simulink library "xbsIndex_r4"  (Simulink 7.1)
(part 2 of 9)

      | patch([3 131 131 3 3 ],[0 0 165 165 0 ],[7.700000e-001 8.200000e-001 9.100000e-001 ]);
      | plot([3 131 131 3 3 ],[0 0 165 165 0 ]);
      | 
      | 
      | patch([24.725 52.18 71.18 90.18 109.18 71.18 43.725 24.725 ],[103.09 103.09 122.09 103.09 122.09 122.09 122.09 103.09 ],[1 1 1 ]);
      | patch([43.725 71.18 52.18 24.725 43.725 ],[84.09 84.09 103.09 103.09 84.09 ],[0.931 0.946 0.973 ]);
      | patch([24.725 52.18 71.18 43.725 24.725 ],[65.09 65.09 84.09 84.09 65.09 ],[1 1 1 ]);
      | patch([43.725 109.18 90.18 71.18 52.18 24.725 43.725 ],[46.09 46.09 65.09 46.09 65.09 65.09 46.09 ],[0.931 0.946 0.973 ]);
      | fprintf('','COMMENT: end icon graphics');
      | fprintf('','COMMENT: begin icon text');
      | color('black');port_label('input',1,'  a_tvalid  ');
      | color('black');port_label('input',2,'  a_tdata_imag  ');
      | color('black');port_label('input',3,'  a_tdata_real  ');
      | color('black');port_label('input',4,'  b_tvalid  ');
      | color('black');port_label('input',5,'  b_tdata_imag  ');
      | color('black');port_label('input',6,'  b_tdata_real  ');
      | color('black');port_label('output',1,'  dout_tvalid  ');
      | color('black');port_label('output',2,'  dout_tdata_imag  ');
      | color('black');port_label('output',3,'  dout_tdata_real  ');
      | fprintf('','COMMENT: end icon text');
  "Complex Multiplier 5.0 " : S-Function  LoadFcn=xlBlockLoadCallback(gcbh);  FunctionName=sysgen  Parameters=ptable_  EnableBusSupport=off  mask(Xilinx Complex Multiplier 5.0  Block){hasatlast_sgadvanced=, hasatlast=off, hasatuser_sgadvanced=, hasatuser=off, atuserwidth=1, hasbtlast_sgadvanced=, hasbtlast=off, hasbtuser_sgadvanced=, hasbtuser=off, btuserwidth=1, multtype_sgadvanced=, multtype=Use_Mults, optimizegoal_sgadvanced=, optimizegoal=Resources, flowcontrol_sgadvanced=, flowcontrol=NonBlocking, outputwidth=33, roundmode_sgadvanced=, roundmode=Truncate, hasctrltlast_sgadvanced=, hasctrltlast=off, hasctrltuser_sgadvanced=, hasctrltuser=off, ctrltuserwidth=1, outtlastbehv=Null, latencyconfig=Automatic, minimumlatency=15, aclken_sgadvanced=, aclken=off, aresetn_sgadvanced=, aresetn=off, trim_axipin_name=on, aportwidth=63, bportwidth=63, ip_name=Complex Multiplier, ip_version=5.0, dsptool_ready=true, ipcore_usecache=true, ipcore_useipmodelcache=true, ipcore_verbose=false, ipcore_latency_parameter='minimumlatency', wrapper_available=true, port_translation_map={ 'aclken' => 'en', 'aresetn' => 'rst'}, structural_sim=false, has_advanced_control=0, sggui_pos=-1,-1,-1,-1, block_type=cmpy_v5_0, block_version=, sg_icon_stat=135,165,6,3,white,blue,0,7e63527f,right,,[2 2 2 3 3 3 ],[4 4 4 ], sg_mask_display=|, sg_list_contents=, sg_blockgui_xml=}
      mask sg_mask_display=|
      | fprintf('','COMMENT: begin icon graphics');
      | patch([0 0 3 3 ],[154 86 86 154 ],[6.025000e-001 6.400000e-001 7.075000e-001 ]);
      | patch([0 0 3 3 ],[79 11 11 79 ],[4.350000e-001 4.600000e-001 5.050000e-001 ]);
      | patch([132 132 135 135 ],[154 6 6 154 ],[2.675000e-001 2.800000e-001 3.025000e-001 ]);
      | patch([3 131 131 3 3 ],[0 0 165 165 0 ],[7.700000e-001 8.200000e-001 9.100000e-001 ]);
      | plot([3 131 131 3 3 ],[0 0 165 165 0 ]);
      |
      |
      | patch([24.725 52.18 71.18 90.18 109.18 71.18 43.725 24.725 ],[103.09 103.09 122.09 103.09 122.09 122.09 122.09 103.09 ],[1 1 1 ]);
      | patch([43.725 71.18 52.18 24.725 43.725 ],[84.09 84.09 103.09 103.09 84.09 ],[0.931 0.946 0.973 ]);
      | patch([24.725 52.18 71.18 43.725 24.725 ],[65.09 65.09 84.09 84.09 65.09 ],[1 1 1 ]);
      | patch([43.725 109.18 90.18 71.18 52.18 24.725 43.725 ],[46.09 46.09 65.09 46.09 65.09 65.09 46.09 ],[0.931 0.946 0.973 ]);
      | fprintf('','COMMENT: end icon graphics');
      | fprintf('','COMMENT: begin icon text');
      | color('black');port_label('input',1,'  a_tvalid  ');
      | color('black');port_label('input',2,'  a_tdata_imag  ');
      | color('black');port_label('input',3,'  a_tdata_real  ');
      | color('black');port_label('input',4,'  b_tvalid  ');
      | color('black');port_label('input',5,'  b_tdata_imag  ');
      | color('black');port_label('input',6,'  b_tdata_real  ');
      | color('black');port_label('output',1,'  dout_tvalid  ');
      | color('black');port_label('output',2,'  dout_tdata_imag  ');
      | color('black');port_label('output',3,'  dout_tdata_real  ');
      | fprintf('','COMMENT: end icon text');
      mask prompts: hasatlast_sgadvanced ""; hasatlast "Has TLAST"; hasatuser_sgadvanced ""; hasatuser "Has TUSER"; atuserwidth "TUSER Width"; hasbtlast_sgadvanced ""; hasbtlast "Has TLAST"; hasbtuser_sgadvanced ""; hasbtuser "Has TUSER"; btuserwidth "TUSER Width"; multtype_sgadvanced ""; multtype ""; optimizegoal_sgadvanced ""; optimizegoal ""; flowcontrol_sgadvanced ""; flowcontrol ""; outputwidth "Output Width"; roundmode_sgadvanced ""; roundmode ""; hasctrltlast_sgadvanced ""; hasctrltlast "Has TLAST"; hasctrltuser_sgadvanced ""; hasctrltuser "Has TUSER"; ctrltuserwidth "TUSER Width"; outtlastbehv "TLAST Behavior"; latencyconfig "Latency Configuration"; minimumlatency "Minimum Latency"; aclken_sgadvanced ""; aresetn_sgadvanced ""; trim_axipin_name "Display shortened port names"; aportwidth ""; bportwidth ""; ip_name ""; ip_version ""; dsptool_ready ""; ipcore_usecache ""; ipcore_useipmodelcache ""; ipcore_verbose ""; ipcore_latency_parameter ""; wrapper_available ""; port_translation_map ""; structural_sim ""; has_advanced_control ""; sggui_pos ""; block_type ""; block_version ""; sg_icon_stat ""; sg_mask_display ""; sg_list_contents ""; sg_blockgui_xml ""
      mask help: Xilinx Complex Multiplier 5.0
      mask init:
      | try
      |   tmp_gcb = gcb;
      |   tmp_gcbh = gcbh;
      |   if (strcmp('SysGenIndex',get_param(bdroot(tmp_gcbh),'tag')) && ~isempty(regexp(bdroot(tmp_gcb), '^xbs', 'once')))
      |     return;
      |   end;
      |   xlMungeMaskParams;
      |   block_config = 'sysgen:coregenimport_config';
      | 
      |   block_type='cmpy_v5_0';
      | 
      |   serialized_declarations = '{''aclken''=>''Bool'',''aportwidth''=>''String'',''aresetn''=>''Bool'',''atuserwidth''=>''Int'',''bportwidth''=>''String'',''btuserwidth''=>''Int'',''ctrltuserwidth''=>''Int'',''dsptool_ready''=>''Bool'',''flowcontrol''=>''String'',''hasatlast''=>''Bool'',''hasatuser''=>''Bool'',''hasbtlast''=>''Bool'',''hasbtuser''=>''Bool'',''hasctrltlast''=>''Bool'',''hasctrltuser''=>''Bool'',''ip_name''=>''String'',''ip_version''=>''String'',''ipcore_latency_parameter''=>''String'',''ipcore_usecache''=>''Bool'',''ipcore_useipmodelcache''=>''Bool'',''ipcore_verbose''=>''Bool'',''latencyconfig''=>''String'',''minimumlatency''=>''Int'',''multtype''=>''String'',''optimizegoal''=>''String'',''outputwidth''=>''Int'',''outtlastbehv''=>''String'',''port_translation_map''=>''String'',''roundmode''=>''String'',''structural_sim''=>''Bool'',''trim_axipin_name''=>''Int'',''wrapper_available''=>''Bool'',''block_type''=>''String''}';
      |   ptable_ = xlblockprep(get_param(tmp_gcb, 'MaskWSVariables'));
      |   try
      |     xlBlockMoveCallback(tmp_gcbh);
      |   catch 
      |      clear global xl_updateicon_recursion_guard;
      |   end;
      | catch
      |   global dbgsysgen;
      |   if(~isempty(dbgsysgen) && dbgsysgen)
      |     e = regexprep(lasterr, '\n', '\nError: ');
      |     disp(['Error: While running MaskInit code on block ' tmp_gcb ': ' e]);
      |     error(e);
      |   end
      | end
      settings: CopyFcn=xlBlockMoveCallback(gcbh);  DeleteFcn=xlDestroyGui(gcbh);  ModelCloseFcn=xlDestroyGui(gcbh);  PreSaveFcn=xlBlockPreSaveCallback(gcbh);  PostSaveFcn=xlBlockPostSaveCallback(gcbh);  DestroyFcn=xlDestroyGui(gcbh);  OpenFcn=xlOpenGui(gcbh, 'cmpy_v5_0_gui.xml', @xlipmagiccallback_pass_evaluate_params, @xlipmagicaction)  CloseFcn=xlDestroyGui(gcbh);  MoveFcn=xlBlockMoveCallback(gcbh);
      mask Help: eval('');xlDoc('-book','sysgen','-topic','Complex_Multiplier_5_0');
      mask StyleString: edit,checkbox,edit,checkbox,edit,edit,checkbox,edit,checkbox,edit,edit,popup(Use_Mults|Use_LUTs),edit,popup(Resources|Performance),edit,popup(Blocking|NonBlocking),edit,edit,popup(Truncate|Random_Rounding),edit,checkbox,edit,checkbox,edit,popup(Null|Pass_A_TLAST|Pass_B_TLAST|Pass_CTRL_TLAST|OR_all_TLASTs|AND_all_TLASTs),popup(Automatic|Manual),edit,edit,checkbox,edit,checkbox,checkbox,edit,edit,edit,edit,edit,edit,edit,edit,edit,edit,edit,edit,edit,edit,edit,edit,edit,edit,edit,edit
      mask Display:
      | fprintf('','COMMENT: begin icon graphics');
      | patch([0 0 3 3 ],[154 86 86 154 ],[6.025000e-001 6.400000e-001 7.075000e-001 ]);
      | patch([0 0 3 3 ],[79 11 11 79 ],[4.350000e-001 4.600000e-001 5.050000e-001 ]);
      | patch([132 132 135 135 ],[154 6 6 154 ],[2.675000e-001 2.800000e-001 3.025000e-001 ]);
      | patch([3 131 131 3 3 ],[0 0 165 165 0 ],[7.700000e-001 8.200000e-001 9.100000e-001 ]);
      | plot([3 131 131 3 3 ],[0 0 165 165 0 ]);
      | 
      | 
      | patch([24.725 52.18 71.18 90.18 109.18 71.18 43.725 24.725 ],[103.09 103.09 122.09 103.09 122.09 122.09 122.09 103.09 ],[1 1 1 ]);
      | patch([43.725 71.18 52.18 24.725 43.725 ],[84.09 84.09 103.09 103.09 84.09 ],[0.931 0.946 0.973 ]);
      | patch([24.725 52.18 71.18 43.725 24.725 ],[65.09 65.09 84.09 84.09 65.09 ],[1 1 1 ]);
      | patch([43.725 109.18 90.18 71.18 52.18 24.725 43.725 ],[46.09 46.09 65.09 46.09 65.09 65.09 46.09 ],[0.931 0.946 0.973 ]);
      | fprintf('','COMMENT: end icon graphics');
      | fprintf('','COMMENT: begin icon text');
      | color('black');port_label('input',1,'  a_tvalid  ');
      | color('black');port_label('input',2,'  a_tdata_imag  ');
      | color('black');port_label('input',3,'  a_tdata_real  ');
      | color('black');port_label('input',4,'  b_tvalid  ');
      | color('black');port_label('input',5,'  b_tdata_imag  ');
      | color('black');port_label('input',6,'  b_tdata_real  ');
      | color('black');port_label('output',1,'  dout_tvalid  ');
      | color('black');port_label('output',2,'  dout_tdata_imag  ');
      | color('black');port_label('output',3,'  dout_tdata_real  ');
      | fprintf('','COMMENT: end icon text');
  Concat : S-Function  LoadFcn=xlBlockLoadCallback(gcbh);  FunctionName=sysgen  Parameters=ptable_  EnableBusSupport=off  mask(Xilinx Bus Concatenator Block){infoedit=Concatenates two or more inputs.  Output will be cast to an unsigned value with the binary point at zero., num_inputs=2, dbl_ovrd_sgadvanced=, dbl_ovrd=off, has_advanced_control=0, sggui_pos=-1,-1,-1,-1, block_type=concat, block_version=, sg_icon_stat=60,60,2,1,white,blue,0,16398980,right,,[ ],[ ], sg_mask_display=|, sg_list_contents=, sg_blockgui_xml=}
      mask sg_mask_display=|
      | fprintf('','COMMENT: begin icon graphics');
      | patch([0 60 60 0 0 ],[0 0 60 60 0 ],[0.77 0.82 0.91 ]);
      | plot([0 60 60 0 0 ],[0 0 60 60 0 ]);
      | patch([12.2 23.76 31.76 39.76 47.76 31.76 20.2 12.2 ],[38.88 38.88 46.88 38.88 46.88 46.88 46.88 38.88 ],[1 1 1 ]);
      | patch([20.2 31.76 23.76 12.2 20.2 ],[30.88 30.88 38.88 38.88 30.88 ],[0.931 0.946 0.973 ]);
      | patch([12.2 23.76 31.76 20.2 12.2 ],[22.88 22.88 30.88 30.88 22.88 ],[1 1 1 ]);
      | patch([20.2 47.76 39.76 31.76 23.76 12.2 20.2 ],[14.88 14.88 22.88 14.88 22.88 22.88 14.88 ],[0.931 0.946 0.973 ]);
      | fprintf('','COMMENT: end icon graphics');
      | fprintf('','COMMENT: begin icon text');
      | color('black');port_label('input',1,'hi');
      | color('black');port_label('input',2,'lo');
      |
      | color('black');disp('\fontsize{20}\}','texmode','on');
      | fprintf('','COMMENT: end icon text');
      mask prompts: infoedit ""; num_inputs "Number of inputs"; dbl_ovrd_sgadvanced ""; dbl_ovrd "Override with doubles"; has_advanced_control ""; sggui_pos ""; block_type ""; block_version ""; sg_icon_stat ""; sg_mask_display ""; sg_list_contents ""; sg_blockgui_xml ""
      mask help: Concatenates two or more inputs. Output will be cast to an unsigned value with the binary point at zero.
      mask init:
      | try
      |   tmp_gcb = gcb;
      |   tmp_gcbh = gcbh;
      |   if (strcmp('SysGenIndex',get_param(bdroot(tmp_gcbh),'tag')) && ~isempty(regexp(bdroot(tmp_gcb), '^xbs', 'once')))
      |     return;
      |   end;
      |   xlMungeMaskParams;
      |   block_config = 'sysgen_blockset:Concat_config';
      | 
      |   block_type='concat';
      | 
      |   serialized_declarations = '{''num_inputs''=>''Int'',''sim_engine''=>''Int'',''sysgen_root''=>''String'',''block_type''=>''String''}';
      |   xlconcat_init();
      |   ptable_ = xlblockprep(get_param(tmp_gcb, 'MaskWSVariables'));
      |   try
      |     xlBlockMoveCallback(tmp_gcbh);
      |   catch 
      |      clear global xl_updateicon_recursion_guard;
      |   end;
      | catch
      |   global dbgsysgen;
      |   if(~isempty(dbgsysgen) && dbgsysgen)
      |     e = regexprep(lasterr, '\n', '\nError: ');
      |     disp(['Error: While running MaskInit code on block ' tmp_gcb ': ' e]);
      |     error(e);
      |   end
      | end
      settings: CopyFcn=xlBlockMoveCallback(gcbh);  DeleteFcn=xlDestroyGui(gcbh);  ModelCloseFcn=xlDestroyGui(gcbh);  PreSaveFcn=xlBlockPreSaveCallback(gcbh);  PostSaveFcn=xlBlockPostSaveCallback(gcbh);  DestroyFcn=xlDestroyGui(gcbh);  OpenFcn=xlOpenGui(gcbh, 'concat_gui.xml', @xlmagicenablement, -1)  CloseFcn=xlDestroyGui(gcbh);  MoveFcn=xlBlockMoveCallback(gcbh);
      mask Help: eval('');xlDoc('-book','sysgen','-topic','Concat');
      mask Display:
      | fprintf('','COMMENT: begin icon graphics');
      | patch([0 60 60 0 0 ],[0 0 60 60 0 ],[0.77 0.82 0.91 ]);
      | plot([0 60 60 0 0 ],[0 0 60 60 0 ]);
      | patch([12.2 23.76 31.76 39.76 47.76 31.76 20.2 12.2 ],[38.88 38.88 46.88 38.88 46.88 46.88 46.88 38.88 ],[1 1 1 ]);
      | patch([20.2 31.76 23.76 12.2 20.2 ],[30.88 30.88 38.88 38.88 30.88 ],[0.931 0.946 0.973 ]);
      | patch([12.2 23.76 31.76 20.2 12.2 ],[22.88 22.88 30.88 30.88 22.88 ],[1 1 1 ]);
      | patch([20.2 47.76 39.76 31.76 23.76 12.2 20.2 ],[14.88 14.88 22.88 14.88 22.88 22.88 14.88 ],[0.931 0.946 0.973 ]);
      | fprintf('','COMMENT: end icon graphics');
      | fprintf('','COMMENT: begin icon text');
      | color('black');port_label('input',1,'hi');
      | color('black');port_label('input',2,'lo');
      | 
      | color('black');disp('\fontsize{20}\}','texmode','on');
      | fprintf('','COMMENT: end icon text');
  Configurable Subsystem Manager : S-Function  Tag=xcfgMgr  FunctionName=xlpermissive  Parameters=''  EnableBusSupport=off  mask(Xilinx Configurable Subsystem Manager Block){infoedit=Configurable Subsystem Manager, ShowPortLabels=, has_advanced_control=0, sggui_pos=-1,-1,-1,-1, block_type=configurable_subsystem_manager, block_version=, sg_icon_stat=53,51,-1,-1,blue,white,0,07734,right,,[ ],[ ], sg_mask_display=|, sg_list_contents=, sg_blockgui_xml=}
      mask sg_mask_display=|
      | fprintf('','COMMENT: begin icon graphics');
      | patch([0 53 53 0 0 ],[0 0 51 51 0 ],[1 1 1 ]);
      | plot([0 53 53 0 0 ],[0 0 51 51 0 ]);
      | patch([10.425 20.54 27.54 34.54 41.54 27.54 17.425 10.425 ],[32.77 32.77 39.77 32.77 39.77 39.77 39.77 32.77 ],[0.839 0.874 0.937 ]);
      | patch([17.425 27.54 20.54 10.425 17.425 ],[25.77 25.77 32.77 32.77 25.77 ],[0.77 0.82 0.91 ]);
      | patch([10.425 20.54 27.54 17.425 10.425 ],[18.77 18.77 25.77 25.77 18.77 ],[0.839 0.874 0.937 ]);
      | patch([17.425 41.54 34.54 27.54 20.54 10.425 17.425 ],[11.77 11.77 18.77 11.77 18.77 18.77 11.77 ],[0.77 0.82 0.91 ]);
      | fprintf('','COMMENT: end icon graphics');
      | fprintf('','COMMENT: begin icon text');
      | fprintf('','COMMENT: end icon text');
      mask prompts: infoedit ""; ShowPortLabels ""; has_advanced_control ""; sggui_pos ""; block_type ""; block_version ""; sg_icon_stat ""; sg_mask_display ""; sg_list_contents ""; sg_blockgui_xml ""
      mask help: Configurable Subsystem Manager
      mask init:
      | try
      |   tmp_gcb = gcb;
      |   tmp_gcbh = gcbh;
      |   if (strcmp('SysGenIndex',get_param(bdroot(tmp_gcbh),'tag')) && ~isempty(regexp(bdroot(tmp_gcb), '^xbs', 'once')))
      |     return;
      |   end;
      |   xlMungeMaskParams;
      | 
      |   block_type='configurable_subsystem_manager';
      | 
      |   serialized_declarations = '{''block_type''=>''String''}';
      |   ptable_ = xlblockprep(get_param(tmp_gcb, 'MaskWSVariables'));
      |   try
      |     xlBlockMoveCallback(tmp_gcbh);
      |   catch 
      |      clear global xl_updateicon_recursion_guard;
      |   end;
      | catch
      |   global dbgsysgen;
      |   if(~isempty(dbgsysgen) && dbgsysgen)
      |     e = regexprep(lasterr, '\n', '\nError: ');
      |     disp(['Error: While running MaskInit code on block ' tmp_gcb ': ' e]);
      |     error(e);
      |   end
      | end
      settings: AttributesFormatString=Configurable Subsystem\nManager  CopyFcn=xlBlockMoveCallback(gcbh);  DeleteFcn=xlconfig_mgr_callback(gcb, 'DeleteFcn');  OpenFcn=xlconfig_mgr_callback(gcb, 'OpenFcn');  MoveFcn=xlBlockMoveCallback(gcbh);
      mask Help: eval('');xlDoc('-book','sysgen','-topic','Configurable_Subsystem_Manager');
      mask Display:
      | fprintf('','COMMENT: begin icon graphics');
      | patch([0 53 53 0 0 ],[0 0 51 51 0 ],[1 1 1 ]);
      | plot([0 53 53 0 0 ],[0 0 51 51 0 ]);
      | patch([10.425 20.54 27.54 34.54 41.54 27.54 17.425 10.425 ],[32.77 32.77 39.77 32.77 39.77 39.77 39.77 32.77 ],[0.839 0.874 0.937 ]);
      | patch([17.425 27.54 20.54 10.425 17.425 ],[25.77 25.77 32.77 32.77 25.77 ],[0.77 0.82 0.91 ]);
      | patch([10.425 20.54 27.54 17.425 10.425 ],[18.77 18.77 25.77 25.77 18.77 ],[0.839 0.874 0.937 ]);
      | patch([17.425 41.54 34.54 27.54 20.54 10.425 17.425 ],[11.77 11.77 18.77 11.77 18.77 18.77 11.77 ],[0.77 0.82 0.91 ]);
      | fprintf('','COMMENT: end icon graphics');
      | fprintf('','COMMENT: begin icon text');
      | fprintf('','COMMENT: end icon text');
  Constant : S-Function  LoadFcn=xlBlockLoadCallback(gcbh);  FunctionName=sysgen  Parameters=ptable_  EnableBusSupport=off  mask(Xilinx Constant Block Block){const=1, gui_display_data_type=Fixed-point, arith_type_sgadvanced=, arith_type=Signed (2's comp), n_bits=16, bin_pt=14, preci_type_sgadvanced=, preci_type=Single, exp_width=8, frac_width=24, explicit_period_sgadvanced=, explicit_period=off, period=1, dsp48_infoedit=The use of this block for DSP48 instructions is deprecated.  Please use the Opmode block., equ=P=C, opselect_sgadvanced=, opselect=C, inp2_sgadvanced=, inp2=PCIN>>17, opr_sgadvanced=, opr=+, inp1_sgadvanced=, inp1=P, carry_sgadvanced=, carry=CIN, dbl_ovrd_sgadvanced=, dbl_ovrd=off, has_advanced_control=0, sggui_pos=-1,-1,-1,-1, block_type=constant, block_version=, sg_icon_stat=55,26,0,1,white,blue,0,1c72b5be,right,,[ ],[ ], sg_mask_display=|, sg_list_contents=, sg_blockgui_xml=}
      mask sg_mask_display=|
      | fprintf('','COMMENT: begin icon graphics');
      | patch([0 55 55 0 0 ],[0 0 26 26 0 ],[0.77 0.82 0.91 ]);
      | plot([0 55 55 0 0 ],[0 0 26 26 0 ]);
      | patch([20.325 24.66 27.66 30.66 33.66 27.66 23.325 20.325 ],[16.33 16.33 19.33 16.33 19.33 19.33 19.33 16.33 ],[1 1 1 ]);
      | patch([23.325 27.66 24.66 20.325 23.325 ],[13.33 13.33 16.33 16.33 13.33 ],[0.931 0.946 0.973 ]);
      | patch([20.325 24.66 27.66 23.325 20.325 ],[10.33 10.33 13.33 13.33 10.33 ],[1 1 1 ]);
      | patch([23.325 33.66 30.66 27.66 24.66 20.325 23.325 ],[7.33 7.33 10.33 7.33 10.33 10.33 7.33 ],[0.931 0.946 0.973 ]);
      | fprintf('','COMMENT: end icon graphics');
      | fprintf('','COMMENT: begin icon text');
      | color('black');port_label('output',1,'1');
      | fprintf('','COMMENT: end icon text');
      mask prompts: const "Constant value"; gui_display_data_type ""; arith_type_sgadvanced ""; arith_type "Arithmetic type"; n_bits "Number of bits"; bin_pt "Binary point"; preci_type_sgadvanced ""; preci_type ""; exp_width "Exponent width"; frac_width "Fraction width"; explicit_period_sgadvanced ""; explicit_period "Sampled constant"; period "Sample period"; dsp48_infoedit ""; equ "DSP48 operation"; opselect_sgadvanced ""; opselect "Operation select"; inp2_sgadvanced ""; inp2 "Z mux"; opr_sgadvanced ""; opr "Operand"; inp1_sgadvanced ""; inp1 "YX muxes"; carry_sgadvanced ""; carry "Carry input"; dbl_ovrd_sgadvanced ""; dbl_ovrd "Override with doubles"; has_advanced_control ""; sggui_pos ""; block_type ""; block_version ""; sg_icon_stat ""; sg_mask_display ""; sg_list_contents ""; sg_blockgui_xml ""
      mask help: Xilinx Constant Block
      mask init:
      | try
      |   tmp_gcb = gcb;
      |   tmp_gcbh = gcbh;
      |   if (strcmp('SysGenIndex',get_param(bdroot(tmp_gcbh),'tag')) && ~isempty(regexp(bdroot(tmp_gcb), '^xbs', 'once')))
      |     return;
      |   end;
      |   xlMungeMaskParams;
      |   block_config = 'sysgen_blockset:Constant_config';
      | 
      |   block_type='constant';
      | 
      |   serialized_declarations = '{''arith_type''=>''Int'',''bin_pt''=>''Int'',''carry''=>''Int'',''const''=>''Double'',''dbl_ovrd''=>''Int'',''exp_width''=>''Int'',''explicit_period''=>''Int'',''frac_width''=>''Int'',''gui_display_data_type''=>''Int'',''inp1''=>''Int'',''inp2''=>''Int'',''n_bits''=>''Int'',''opr''=>''Int'',''opselect''=>''Int'',''period''=>''Double'',''preci_type''=>''Int'',''block_type''=>''String''}';
      |   xlconstant_init();
      |   ptable_ = xlblockprep(get_param(tmp_gcb, 'MaskWSVariables'));
      |   try
      |     xlBlockMoveCallback(tmp_gcbh);
      |   catch 
      |      clear global xl_updateicon_recursion_guard;
      |   end;
      | catch
      |   global dbgsysgen;
      |   if(~isempty(dbgsysgen) && dbgsysgen)
      |     e = regexprep(lasterr, '\n', '\nError: ');
      |     disp(['Error: While running MaskInit code on block ' tmp_gcb ': ' e]);
      |     error(e);
      |   end
      | end
      settings: CopyFcn=xlBlockMoveCallback(gcbh);  DeleteFcn=xlDestroyGui(gcbh);  ModelCloseFcn=xlDestroyGui(gcbh);  PreSaveFcn=xlBlockPreSaveCallback(gcbh);  PostSaveFcn=xlBlockPostSaveCallback(gcbh);  DestroyFcn=xlDestroyGui(gcbh);  OpenFcn=xlOpenGui(gcbh, 'constant_gui.xml', @constantenablement, @constantaction)  CloseFcn=xlDestroyGui(gcbh);  MoveFcn=xlBlockMoveCallback(gcbh);
      mask Help: eval('');xlDoc('-book','sysgen','-topic','Constant');
      mask StyleString: edit,popup(Boolean|Fixed-point|Floating-point),edit,popup(Boolean|Signed (2's comp)|Unsigned|DSP48 Instruction|Floating-point),edit,edit,edit,popup(Single|Double|Custom),edit,edit,edit,checkbox,edit,edit,edit,edit,popup(C + A*B|PCIN + A*B|P + A*B|A * B|C + A:B|C - A:B|C|Custom),edit,popup(0|PCIN|P|C|PCIN>>17|P>>17),edit,popup(+|-),edit,popup(0|P|A:B|A*B|C|P+C|A:B+C),edit,popup(0|1|CIN|~SIGN(P or PCIN)|~SIGN(A*B or A:B)|~SIGND(A*B or A:B)),edit,checkbox,edit,edit,edit,edit,edit,edit,edit,edit
      mask Display:
      | fprintf('','COMMENT: begin icon graphics');
      | patch([0 55 55 0 0 ],[0 0 26 26 0 ],[0.77 0.82 0.91 ]);
      | plot([0 55 55 0 0 ],[0 0 26 26 0 ]);
      | patch([20.325 24.66 27.66 30.66 33.66 27.66 23.325 20.325 ],[16.33 16.33 19.33 16.33 19.33 19.33 19.33 16.33 ],[1 1 1 ]);
      | patch([23.325 27.66 24.66 20.325 23.325 ],[13.33 13.33 16.33 16.33 13.33 ],[0.931 0.946 0.973 ]);
      | patch([20.325 24.66 27.66 23.325 20.325 ],[10.33 10.33 13.33 13.33 10.33 ],[1 1 1 ]);
      | patch([23.325 33.66 30.66 27.66 24.66 20.325 23.325 ],[7.33 7.33 10.33 7.33 10.33 10.33 7.33 ],[0.931 0.946 0.973 ]);
      | fprintf('','COMMENT: end icon graphics');
      | fprintf('','COMMENT: begin icon text');
      | color('black');port_label('output',1,'1');
      | fprintf('','COMMENT: end icon text');
  Convert : S-Function  LoadFcn=xlBlockLoadCallback(gcbh);  FunctionName=sysgen  Parameters=ptable_  EnableBusSupport=off  mask(Xilinx Type Converter Block){infoedit=Hardware notes: rounding and saturating require hardware resources; truncating and wrapping do not., gui_display_data_type_sgadvanced=, gui_display_data_type=Fixed-point, arith_type_sgadvanced=, arith_type=Signed  (2's comp), n_bits=16, bin_pt=14, float_type_sgadvanced=, float_type=Single, exp_bits=8, fraction_bits=24, quantization_sgadvanced=, quantization=Truncate, overflow_sgadvanced=, overflow=Wrap, en_sgadvanced=, en=off, latency=0, dbl_ovrd_sgadvanced=, dbl_ovrd=off, pipeline_sgadvanced=, pipeline=off, xl_use_area_sgadvanced=, xl_use_area=off, xl_area=[0,0,0,0,0,0,0], has_advanced_control=0, sggui_pos=-1,-1,-1,-1, block_type=convert, block_version=, sg_icon_stat=45,30,1,1,white,blue,0,edca21da,right,,[ ],[ ], sg_mask_display=|, sg_list_contents=, sg_blockgui_xml=}
      mask sg_mask_display=|
      | fprintf('','COMMENT: begin icon graphics');
      | patch([0 45 45 0 0 ],[0 0 30 30 0 ],[0.77 0.82 0.91 ]);
      | plot([0 45 45 0 0 ],[0 0 30 30 0 ]);
      | patch([13.1 18.88 22.88 26.88 30.88 22.88 17.1 13.1 ],[19.44 19.44 23.44 19.44 23.44 23.44 23.44 19.44 ],[1 1 1 ]);
      | patch([17.1 22.88 18.88 13.1 17.1 ],[15.44 15.44 19.44 19.44 15.44 ],[0.931 0.946 0.973 ]);
      | patch([13.1 18.88 22.88 17.1 13.1 ],[11.44 11.44 15.44 15.44 11.44 ],[1 1 1 ]);
      | patch([17.1 30.88 26.88 22.88 18.88 13.1 17.1 ],[7.44 7.44 11.44 7.44 11.44 11.44 7.44 ],[0.931 0.946 0.973 ]);
      | fprintf('','COMMENT: end icon graphics');
      | fprintf('','COMMENT: begin icon text');
      |
      | color('black');port_label('output',1,'cast');
      | fprintf('','COMMENT: end icon text');
      mask prompts: infoedit ""; gui_display_data_type_sgadvanced ""; gui_display_data_type ""; arith_type_sgadvanced ""; arith_type "Arithmetic type"; n_bits "Number of bits"; bin_pt "Binary point"; float_type_sgadvanced ""; float_type ""; exp_bits "Exponent width"; fraction_bits "Fraction width"; quantization_sgadvanced ""; overflow_sgadvanced ""; en_sgadvanced ""; en "Provide enable port"; dbl_ovrd_sgadvanced ""; dbl_ovrd "Override with doubles"; pipeline_sgadvanced ""; pipeline "Pipeline for maximum performance"; xl_use_area_sgadvanced ""; xl_use_area "Define FPGA area for resource estimation"; xl_area "FPGA area [slices, FFs, BRAMs, LUTs, IOBs, emb. mults, TBUFs]"; has_advanced_control ""; sggui_pos ""; block_type ""; block_version ""; sg_icon_stat ""; sg_mask_display ""; sg_list_contents ""; sg_blockgui_xml ""
      mask help: Hardware notes: rounding and saturating require hardware resources; truncating and wrapping do not.
      mask init:
      | try
      |   tmp_gcb = gcb;
      |   tmp_gcbh = gcbh;
      |   if (strcmp('SysGenIndex',get_param(bdroot(tmp_gcbh),'tag')) && ~isempty(regexp(bdroot(tmp_gcb), '^xbs', 'once')))
      |     return;
      |   end;
      |   xlMungeMaskParams;
      |   block_config = 'sysgen_blockset:Convert_config';
      | 
      |   block_type='convert';
      | 
      |   serialized_declarations = '{''arith_type''=>''Int'',''bin_pt''=>''Int'',''en''=>''Int'',''exp_bits''=>''Int'',''float_type''=>''Int'',''fraction_bits''=>''Int'',''gui_display_data_type''=>''Int'',''latency''=>''Int'',''n_bits''=>''Int'',''overflow''=>''Int'',''pipeline''=>''Int'',''quantization''=>''Int'',''sim_engine''=>''Int'',''sysgen_root''=>''String'',''block_type''=>''String''}';
      |   xlconvert_init();
      |   ptable_ = xlblockprep(get_param(tmp_gcb, 'MaskWSVariables'));
      |   try
      |     xlBlockMoveCallback(tmp_gcbh);
      |   catch 
      |      clear global xl_updateicon_recursion_guard;
      |   end;
      | catch
      |   global dbgsysgen;
      |   if(~isempty(dbgsysgen) && dbgsysgen)
      |     e = regexprep(lasterr, '\n', '\nError: ');
      |     disp(['Error: While running MaskInit code on block ' tmp_gcb ': ' e]);
      |     error(e);
      |   end
      | end
      settings: CopyFcn=xlBlockMoveCallback(gcbh);  DeleteFcn=xlDestroyGui(gcbh);  ModelCloseFcn=xlDestroyGui(gcbh);  PreSaveFcn=xlBlockPreSaveCallback(gcbh);  PostSaveFcn=xlBlockPostSaveCallback(gcbh);  DestroyFcn=xlDestroyGui(gcbh);  OpenFcn=xlOpenGui(gcbh, 'convert_gui.xml', @convertenablement, @convertaction)  CloseFcn=xlDestroyGui(gcbh);  MoveFcn=xlBlockMoveCallback(gcbh);
      mask Help: eval('');xlDoc('-book','sysgen','-topic','Convert');
      mask StyleString: edit,edit,popup(Boolean|Fixed-point|Floating-point),edit,popup(Boolean|Signed  (2's comp)|Unsigned|Floating-point),edit,edit,edit,popup(Single|Double|Custom),edit,edit,edit,popup(Truncate|Round  (unbiased: +/- Inf)|Round  (unbiased: Even Values)),edit,popup(Wrap|Saturate|Flag as error),edit,checkbox,edit,edit,checkbox,edit,checkbox,edit,checkbox,edit,edit,edit,edit,edit,edit,edit,edit,edit
      mask Display:
      | fprintf('','COMMENT: begin icon graphics');
      | patch([0 45 45 0 0 ],[0 0 30 30 0 ],[0.77 0.82 0.91 ]);
      | plot([0 45 45 0 0 ],[0 0 30 30 0 ]);
      | patch([13.1 18.88 22.88 26.88 30.88 22.88 17.1 13.1 ],[19.44 19.44 23.44 19.44 23.44 23.44 23.44 19.44 ],[1 1 1 ]);
      | patch([17.1 22.88 18.88 13.1 17.1 ],[15.44 15.44 19.44 19.44 15.44 ],[0.931 0.946 0.973 ]);
      | patch([13.1 18.88 22.88 17.1 13.1 ],[11.44 11.44 15.44 15.44 11.44 ],[1 1 1 ]);
      | patch([17.1 30.88 26.88 22.88 18.88 13.1 17.1 ],[7.44 7.44 11.44 7.44 11.44 11.44 7.44 ],[0.931 0.946 0.973 ]);
      | fprintf('','COMMENT: end icon graphics');
      | fprintf('','COMMENT: begin icon text');
      | 
      | color('black');port_label('output',1,'cast');
      | fprintf('','COMMENT: end icon text');
  "Convolution Encoder 7.0 " : S-Function  LoadFcn=xlBlockLoadCallback(gcbh);  FunctionName=sysgen  Parameters=ptable_  EnableBusSupport=off  mask(Xilinx Convolution Encoder 7.0  Block){input_rate=1, output_rate=2, punctured_sgadvanced=, punctured=off, dual_output_sgadvanced=, dual_output=off, puncture_code0='0', puncture_code1='0', constraint_length=7, convolution_code0='1001111', convolution_code1='1101101', convolution_code2='0000011', convolution_code3='0000011', convolution_code4='0000011', convolution_code5='0000011', convolution_code6='0000011', nd_sgadvanced=, nd=off, rfd_sgadvanced=, rfd=off, fd_in_sgadvanced=, fd_in=off, rffd_sgadvanced=, rffd=off, rdy_sgadvanced=, rdy=off, synchronous_clear_sgadvanced=, synchronous_clear=off, ce_sgadvanced=, ce=off, ip_name=Convolution Encoder, ip_version=7.0, dsptool_ready=false, ipcore_usecache=true, ipcore_useipmodelcache=true, wrapper_available=true, port_translation_map={ 'ce' => 'en', 'sclr' => 'rst'}, structural_sim=true, ipcore_do_not_force_period=true, has_advanced_control=0, sggui_pos=-1,-1,-1,-1, block_type=convolution_v7_0, block_version=, sg_icon_stat=95,142,1,1,white,blue,0,ad834320,right,,[ ],[ ], sg_mask_display=|, sg_list_contents=, sg_blockgui_xml=}
      mask sg_mask_display=|
      | fprintf('','COMMENT: begin icon graphics');
      | patch([0 95 95 0 0 ],[0 0 142 142 0 ],[0.77 0.82 0.91 ]);
      | plot([0 95 95 0 0 ],[0 0 142 142 0 ]);
      | patch([18.075 36.86 49.86 62.86 75.86 49.86 31.075 18.075 ],[85.43 85.43 98.43 85.43 98.43 98.43 98.43 85.43 ],[1 1 1 ]);
      | patch([31.075 49.86 36.86 18.075 31.075 ],[72.43 72.43 85.43 85.43 72.43 ],[0.931 0.946 0.973 ]);
      | patch([18.075 36.86 49.86 31.075 18.075 ],[59.43 59.43 72.43 72.43 59.43 ],[1 1 1 ]);
      | patch([31.075 75.86 62.86 49.86 36.86 18.075 31.075 ],[46.43 46.43 59.43 46.43 59.43 59.43 46.43 ],[0.931 0.946 0.973 ]);
      | fprintf('','COMMENT: end icon graphics');
      | fprintf('','COMMENT: begin icon text');
      | color('black');port_label('input',1,'data_in');
      | color('black');port_label('output',1,'data_out_v');
      | fprintf('','COMMENT: end icon text');
      mask prompts: input_rate "Input Rate"; output_rate "Output Rate"; punctured_sgadvanced ""; dual_output_sgadvanced ""; dual_output "Dual Output"; puncture_code0 "Puncture Code0"; puncture_code1 "Puncture Code1"; constraint_length "Constraint Length"; convolution_code0 "Convolution Code0"; convolution_code1 "Convolution Code1"; convolution_code2 "Convolution Code2"; convolution_code3 "Convolution Code3"; convolution_code4 "Convolution Code4"; convolution_code5 "Convolution Code5"; convolution_code6 "Convolution Code6"; nd_sgadvanced ""; rfd_sgadvanced ""; fd_in_sgadvanced ""; rffd_sgadvanced ""; rdy_sgadvanced ""; synchronous_clear_sgadvanced ""; synchronous_clear "SCLR"; ce_sgadvanced ""; ip_name ""; ip_version ""; dsptool_ready ""; ipcore_usecache ""; ipcore_useipmodelcache ""; wrapper_available ""; port_translation_map ""; structural_sim ""; ipcore_do_not_force_period ""; has_advanced_control ""; sggui_pos ""; block_type ""; block_version ""; sg_icon_stat ""; sg_mask_display ""; sg_list_contents ""; sg_blockgui_xml ""
      mask help: Xilinx Convolution Encoder 7.0
      mask init:
      | try
      |   tmp_gcb = gcb;
      |   tmp_gcbh = gcbh;
      |   if (strcmp('SysGenIndex',get_param(bdroot(tmp_gcbh),'tag')) && ~isempty(regexp(bdroot(tmp_gcb), '^xbs', 'once')))
      |     return;
      |   end;
      |   xlMungeMaskParams;
      |   block_config = 'sysgen:coregenimport_config';
      | 
      |   block_type='convolution_v7_0';
      | 
      |   serialized_declarations = '{''ce''=>''Bool'',''constraint_length''=>''String'',''convolution_code0''=>''String'',''convolution_code1''=>''String'',''convolution_code2''=>''String'',''convolution_code3''=>''String'',''convolution_code4''=>''String'',''convolution_code5''=>''String'',''convolution_code6''=>''String'',''dsptool_ready''=>''Bool'',''dual_output''=>''Bool'',''fd_in''=>''Bool'',''input_rate''=>''Int'',''ip_name''=>''String'',''ip_version''=>''String'',''ipcore_do_not_force_period''=>''Bool'',''ipcore_usecache''=>''Bool'',''ipcore_useipmodelcache''=>''Bool'',''nd''=>''Bool'',''output_rate''=>''Int'',''port_translation_map''=>''String'',''puncture_code0''=>''String'',''puncture_code1''=>''String'',''punctured''=>''Bool'',''rdy''=>''Bool'',''rfd''=>''Bool'',''rffd''=>''Bool'',''structural_sim''=>''Bool'',''synchronous_clear''=>''Bool'',''wrapper_available''=>''Bool'',''block_type''=>''String''}';
      |   ptable_ = xlblockprep(get_param(tmp_gcb, 'MaskWSVariables'));
      |   try
      |     xlBlockMoveCallback(tmp_gcbh);
      |   catch 
      |      clear global xl_updateicon_recursion_guard;
      |   end;
      | catch
      |   global dbgsysgen;
      |   if(~isempty(dbgsysgen) && dbgsysgen)
      |     e = regexprep(lasterr, '\n', '\nError: ');
      |     disp(['Error: While running MaskInit code on block ' tmp_gcb ': ' e]);
      |     error(e);
      |   end
      | end
      settings: CopyFcn=xlBlockMoveCallback(gcbh);  DeleteFcn=xlDestroyGui(gcbh);  ModelCloseFcn=xlDestroyGui(gcbh);  PreSaveFcn=xlBlockPreSaveCallback(gcbh);  PostSaveFcn=xlBlockPostSaveCallback(gcbh);  DestroyFcn=xlDestroyGui(gcbh);  OpenFcn=xlOpenGui(gcbh, 'convolution_v7_0_gui.xml', @xlipmagiccallback_pass_evaluate_params, @xlipmagicaction)  CloseFcn=xlDestroyGui(gcbh);  MoveFcn=xlBlockMoveCallback(gcbh);
      mask Help: eval('');xlDoc('-book','sysgen','-topic','Convolution_Encoder_7_0');
      mask StyleString: edit,edit,edit,checkbox,edit,checkbox,edit,edit,popup(3|4|5|6|7|8|9),edit,edit,edit,edit,edit,edit,edit,edit,checkbox,edit,checkbox,edit,checkbox,edit,checkbox,edit,checkbox,edit,checkbox,edit,checkbox,edit,edit,edit,edit,edit,edit,edit,edit,edit,edit,edit,edit,edit,edit,edit,edit,edit
      mask Display:
      | fprintf('','COMMENT: begin icon graphics');
      | patch([0 95 95 0 0 ],[0 0 142 142 0 ],[0.77 0.82 0.91 ]);
      | plot([0 95 95 0 0 ],[0 0 142 142 0 ]);
      | patch([18.075 36.86 49.86 62.86 75.86 49.86 31.075 18.075 ],[85.43 85.43 98.43 85.43 98.43 98.43 98.43 85.43 ],[1 1 1 ]);
      | patch([31.075 49.86 36.86 18.075 31.075 ],[72.43 72.43 85.43 85.43 72.43 ],[0.931 0.946 0.973 ]);
      | patch([18.075 36.86 49.86 31.075 18.075 ],[59.43 59.43 72.43 72.43 59.43 ],[1 1 1 ]);
      | patch([31.075 75.86 62.86 49.86 36.86 18.075 31.075 ],[46.43 46.43 59.43 46.43 59.43 59.43 46.43 ],[0.931 0.946 0.973 ]);
      | fprintf('','COMMENT: end icon graphics');
      | fprintf('','COMMENT: begin icon text');
      | color('black');port_label('input',1,'data_in');
      | color('black');port_label('output',1,'data_out_v');
      | fprintf('','COMMENT: end icon text');
  "Convolution Encoder 8.0 " : S-Function  LoadFcn=xlBlockLoadCallback(gcbh);  FunctionName=sysgen  Parameters=ptable_  EnableBusSupport=off  mask(Xilinx Convolution Encoder 8.0 Block){punctured=off, dual_output=off, input_rate=1, output_rate=2, puncture_code0='0', puncture_code1='0', convolution_code_radix=Binary, constraint_length=7, convolution_code0='1111001', convolution_code1='1011011', convolution_code2='0000000', convolution_code3='0000000', convolution_code4='0000000', convolution_code5='0000000', convolution_code6='0000000', aclken=off, aresetn=off, trim_axipin_name=on, xl_use_area=off, xl_area=[0,0,0,0,0,0,0], ip_name=Convolution Encoder, ip_version=8.0, dsptool_ready=false, ipcore_usecache=true, ipcore_useipmodelcache=true, wrapper_available=true, port_translation_map={ 'aclken' => 'en', 'aresetn' => 'rst' }, structural_sim=true, ipcore_do_not_force_period=true, oldconvolution_code_radix=Binary, has_advanced_control=0, sggui_pos=-1,-1,-1,-1, block_type=convolution_v8_0, block_version=, sg_icon_stat=95,142,3,3,white,blue,0,10535fbb,right,,[2 2 3 ],[2 3 3 ], sg_mask_display=|, sg_list_contents=, sg_blockgui_xml=}
      mask sg_mask_display=|
      | fprintf('','COMMENT: begin icon graphics');
      | patch([0 0 2 2 ],[132 55 55 132 ],[5.466667e-001 5.800000e-001 6.400000e-001 ]);
      | patch([0 0 2 2 ],[42 10 10 42 ],[3.233333e-001 3.400000e-001 3.700000e-001 ]);
      | patch([93 93 95 95 ],[132 100 100 132 ],[5.466667e-001 5.800000e-001 6.400000e-001 ]);
      | patch([93 93 95 95 ],[87 10 10 87 ],[3.233333e-001 3.400000e-001 3.700000e-001 ]);
      | patch([2 92 92 2 2 ],[0 0 142 142 0 ],[7.700000e-001 8.200000e-001 9.100000e-001 ]);
      | plot([2 92 92 2 2 ],[0 0 142 142 0 ]);
      |
      |
      | patch([18.075 36.86 49.86 62.86 75.86 49.86 31.075 18.075 ],[85.43 85.43 98.43 85.43 98.43 98.43 98.43 85.43 ],[1 1 1 ]);
      | patch([31.075 49.86 36.86 18.075 31.075 ],[72.43 72.43 85.43 85.43 72.43 ],[0.931 0.946 0.973 ]);
      | patch([18.075 36.86 49.86 31.075 18.075 ],[59.43 59.43 72.43 72.43 59.43 ],[1 1 1 ]);
      | patch([31.075 75.86 62.86 49.86 36.86 18.075 31.075 ],[46.43 46.43 59.43 46.43 59.43 59.43 46.43 ],[0.931 0.946 0.973 ]);
      | fprintf('','COMMENT: end icon graphics');
      | fprintf('','COMMENT: begin icon text');
      | color('black');port_label('input',1,'  data_tvalid  ');
      | color('black');port_label('input',2,'  data_tdata_data_in  ');
      | color('black');port_label('input',3,'  data_tready  ');
      | color('black');port_label('output',1,'  data_tready  ');
      | color('black');port_label('output',2,'  data_tvalid  ');
      | color('black');port_label('output',3,'  data_tdata_data_out  ');
      | fprintf('','COMMENT: end icon text');
      mask prompts: dual_output "Dual output"; input_rate "Input rate"; output_rate "Output rate"; puncture_code0 "Puncture code0"; puncture_code1 "Puncture code1"; convolution_code_radix "Convolution code radix"; constraint_length "Constraint length"; convolution_code0 "Convolution code0"; convolution_code1 "Convolution code1"; convolution_code2 "Convolution code2"; convolution_code3 "Convolution code3"; convolution_code4 "Convolution code4"; convolution_code5 "Convolution code5"; convolution_code6 "Convolution code6"; trim_axipin_name "Display shortened port names"; xl_use_area "Define FPGA area for resource estimation"; xl_area "FPGA area [slices, FFs, BRAMs, LUTs, IOBs, emb. mults, TBUFs]"; ip_name ""; ip_version ""; dsptool_ready ""; ipcore_usecache ""; ipcore_useipmodelcache ""; wrapper_available ""; port_translation_map ""; structural_sim ""; ipcore_do_not_force_period ""; oldconvolution_code_radix ""; has_advanced_control ""; sggui_pos ""; block_type ""; block_version ""; sg_icon_stat ""; sg_mask_display ""; sg_list_contents ""; sg_blockgui_xml ""
      mask help: Xilinx Convolution Encoder 8.0
      mask init:
      | try
      |   tmp_gcb = gcb;
      |   tmp_gcbh = gcbh;
      |   if (strcmp('SysGenIndex',get_param(bdroot(tmp_gcbh),'tag')) && ~isempty(regexp(bdroot(tmp_gcb), '^xbs', 'once')))
      |     return;
      |   end;
      |   xlMungeMaskParams;
      |   block_config = 'sysgen:coregenimport_config';
      | 
      |   block_type='convolution_v8_0';
      | 
      |   serialized_declarations = '{''aclken''=>''Bool'',''aresetn''=>''Bool'',''constraint_length''=>''String'',''convolution_code0''=>''String'',''convolution_code1''=>''String'',''convolution_code2''=>''String'',''convolution_code3''=>''String'',''convolution_code4''=>''String'',''convolution_code5''=>''String'',''convolution_code6''=>''String'',''convolution_code_radix''=>''String'',''dsptool_ready''=>''Bool'',''dual_output''=>''Bool'',''input_rate''=>''Int'',''ip_name''=>''String'',''ip_version''=>''String'',''ipcore_do_not_force_period''=>''Bool'',''ipcore_usecache''=>''Bool'',''ipcore_useipmodelcache''=>''Bool'',''oldconvolution_code_radix''=>''String'',''output_rate''=>''Int'',''port_translation_map''=>''String'',''puncture_code0''=>''String'',''puncture_code1''=>''String'',''punctured''=>''Bool'',''structural_sim''=>''Bool'',''trim_axipin_name''=>''Int'',''wrapper_available''=>''Bool'',''xl_use_area''=>''Bool'',''block_type''=>''String''}';
      |   ptable_ = xlblockprep(get_param(tmp_gcb, 'MaskWSVariables'));
      |   try
      |     xlBlockMoveCallback(tmp_gcbh);
      |   catch 
      |      clear global xl_updateicon_recursion_guard;
      |   end;
      | catch
      |   global dbgsysgen;
      |   if(~isempty(dbgsysgen) && dbgsysgen)
      |     e = regexprep(lasterr, '\n', '\nError: ');
      |     disp(['Error: While running MaskInit code on block ' tmp_gcb ': ' e]);
      |     error(e);
      |   end
      | end
      settings: CopyFcn=xlBlockMoveCallback(gcbh);  DeleteFcn=xlDestroyGui(gcbh);  ModelCloseFcn=xlDestroyGui(gcbh);  PreSaveFcn=xlBlockPreSaveCallback(gcbh);  PostSaveFcn=xlBlockPostSaveCallback(gcbh);  DestroyFcn=xlDestroyGui(gcbh);  OpenFcn=xlOpenGui(gcbh, 'convolution_v8_0_gui.xml', @convolutionencoder_v8_0_enablement, @convolutionencoder_v8_0_action)  CloseFcn=xlDestroyGui(gcbh);  MoveFcn=xlBlockMoveCallback(gcbh);
      mask Help: eval('');xlDoc('-book','sysgen','-topic','Convolution_Encoder_8_0');
      mask StyleString: checkbox,checkbox,edit,edit,edit,edit,popup(Binary|Octal|Decimal),popup(3|4|5|6|7|8|9),edit,edit,edit,edit,edit,edit,edit,checkbox,checkbox,checkbox,checkbox,edit,edit,edit,edit,edit,edit,edit,edit,edit,edit,edit,edit,edit,edit,edit,edit,edit,edit,edit
      mask Display:
      | fprintf('','COMMENT: begin icon graphics');
      | patch([0 0 2 2 ],[132 55 55 132 ],[5.466667e-001 5.800000e-001 6.400000e-001 ]);
      | patch([0 0 2 2 ],[42 10 10 42 ],[3.233333e-001 3.400000e-001 3.700000e-001 ]);
      | patch([93 93 95 95 ],[132 100 100 132 ],[5.466667e-001 5.800000e-001 6.400000e-001 ]);
      | patch([93 93 95 95 ],[87 10 10 87 ],[3.233333e-001 3.400000e-001 3.700000e-001 ]);
      | patch([2 92 92 2 2 ],[0 0 142 142 0 ],[7.700000e-001 8.200000e-001 9.100000e-001 ]);
      | plot([2 92 92 2 2 ],[0 0 142 142 0 ]);
      | 
      | 
      | patch([18.075 36.86 49.86 62.86 75.86 49.86 31.075 18.075 ],[85.43 85.43 98.43 85.43 98.43 98.43 98.43 85.43 ],[1 1 1 ]);
      | patch([31.075 49.86 36.86 18.075 31.075 ],[72.43 72.43 85.43 85.43 72.43 ],[0.931 0.946 0.973 ]);
      | patch([18.075 36.86 49.86 31.075 18.075 ],[59.43 59.43 72.43 72.43 59.43 ],[1 1 1 ]);
      | patch([31.075 75.86 62.86 49.86 36.86 18.075 31.075 ],[46.43 46.43 59.43 46.43 59.43 59.43 46.43 ],[0.931 0.946 0.973 ]);
      | fprintf('','COMMENT: end icon graphics');
      | fprintf('','COMMENT: begin icon text');
      | color('black');port_label('input',1,'  data_tvalid  ');
      | color('black');port_label('input',2,'  data_tdata_data_in  ');
      | color('black');port_label('input',3,'  data_tready  ');
      | color('black');port_label('output',1,'  data_tready  ');
      | color('black');port_label('output',2,'  data_tvalid  ');
      | color('black');port_label('output',3,'  data_tdata_data_out  ');
      | fprintf('','COMMENT: end icon text');
  "Convolutional Encoder v3_0 " : S-Function  LoadFcn=xlBlockLoadCallback(gcbh);  FunctionName=sysgen  Parameters=ptable_  EnableBusSupport=off  mask(Xilinx Convolutional Encoder Block){clength=3, conv_codes=[7 5 6], rst_sgadvanced=, rst=off, en_sgadvanced=, en=off, dbl_ovrd_sgadvanced=, dbl_ovrd=off, use_rpm_sgadvanced=, use_rpm=off, xl_use_area_sgadvanced=, xl_use_area=off, xl_area=[0,0,0,0,0,0,0], version=3, useCore=, has_advanced_control=0, sggui_pos=-1,-1,-1,-1, block_type=convencoder, block_version=, sg_icon_stat=75,60,-1,-1,white,blue,0,07734,right,,[ ],[ ], sg_mask_display=|, sg_list_contents=, sg_blockgui_xml=}
      mask sg_mask_display=|
      | fprintf('','COMMENT: begin icon graphics');
      | patch([0 75 75 0 0 ],[0 0 60 60 0 ],[0.77 0.82 0.91 ]);
      | plot([0 75 75 0 0 ],[0 0 60 60 0 ]);
      | patch([19.2 30.76 38.76 46.76 54.76 38.76 27.2 19.2 ],[38.88 38.88 46.88 38.88 46.88 46.88 46.88 38.88 ],[1 1 1 ]);
      | patch([27.2 38.76 30.76 19.2 27.2 ],[30.88 30.88 38.88 38.88 30.88 ],[0.931 0.946 0.973 ]);
      | patch([19.2 30.76 38.76 27.2 19.2 ],[22.88 22.88 30.88 30.88 22.88 ],[1 1 1 ]);
      | patch([27.2 54.76 46.76 38.76 30.76 19.2 27.2 ],[14.88 14.88 22.88 14.88 22.88 22.88 14.88 ],[0.931 0.946 0.973 ]);
      | fprintf('','COMMENT: end icon graphics');
      | fprintf('','COMMENT: begin icon text');
      | fprintf('','COMMENT: end icon text');
      mask prompts: clength "Constraint length"; conv_codes "Convolution code array (octal)"; rst_sgadvanced ""; rst "Provide synchronous reset port"; en_sgadvanced ""; en "Provide enable port"; dbl_ovrd_sgadvanced ""; dbl_ovrd "Override with doubles"; use_rpm_sgadvanced ""; use_rpm "Use core placement information"; xl_use_area_sgadvanced ""; xl_use_area "Define FPGA area for resource estimation"; xl_area "FPGA area [slices, FFs, BRAMs, LUTs, IOBs, emb. mults, TBUFs]"; version ""; useCore ""; has_advanced_control ""; sggui_pos ""; block_type ""; block_version ""; sg_icon_stat ""; sg_mask_display ""; sg_list_contents ""; sg_blockgui_xml ""
      mask help: Xilinx Convolutional Encoder
      mask init:
      | try
      |   tmp_gcb = gcb;
      |   tmp_gcbh = gcbh;
      |   if (strcmp('SysGenIndex',get_param(bdroot(tmp_gcbh),'tag')) && ~isempty(regexp(bdroot(tmp_gcb), '^xbs', 'once')))
      |     return;
      |   end;
      |   xlMungeMaskParams;
      |   block_config = 'sysgen_blockset:Removed_config';
      | 
      |   block_type='convencoder';
      | nport = get_param(gcbh, 'ports');
      | nin = nport(1);
      | nout = nport(2);
      | 
      |   serialized_declarations = '{''clength''=>''Int'',''conv_codes''=>''IntVector'',''en''=>''Int'',''rst''=>''Int'',''use_rpm''=>''Int'',''version''=>''Int'',''block_type''=>''String'',''nin''=>''Double'',''nout''=>''Double''}';
      |   ptable_ = xlblockprep(get_param(tmp_gcb, 'MaskWSVariables'));
      |   try
      |     xlBlockMoveCallback(tmp_gcbh);
      |   catch 
      |      clear global xl_updateicon_recursion_guard;
      |   end;
      | catch
      |   global dbgsysgen;
      |   if(~isempty(dbgsysgen) && dbgsysgen)
      |     e = regexprep(lasterr, '\n', '\nError: ');
      |     disp(['Error: While running MaskInit code on block ' tmp_gcb ': ' e]);
      |     error(e);
      |   end
      | end
      settings: CopyFcn=xlBlockMoveCallback(gcbh);  DeleteFcn=xlDestroyGui(gcbh);  ModelCloseFcn=xlDestroyGui(gcbh);  PreSaveFcn=xlBlockPreSaveCallback(gcbh);  PostSaveFcn=xlBlockPostSaveCallback(gcbh);  DestroyFcn=xlDestroyGui(gcbh);  OpenFcn=xlOpenGui(gcbh, 'convencoder_gui.xml', @xlremovedenablement, -1)  CloseFcn=xlDestroyGui(gcbh);  MoveFcn=xlBlockMoveCallback(gcbh);
      mask Help: eval('');xlDoc('-book','sysgen','-topic','Convolutional_Encoder_v3_0');
      mask Display:
      | fprintf('','COMMENT: begin icon graphics');
      | patch([0 75 75 0 0 ],[0 0 60 60 0 ],[0.77 0.82 0.91 ]);
      | plot([0 75 75 0 0 ],[0 0 60 60 0 ]);
      | patch([19.2 30.76 38.76 46.76 54.76 38.76 27.2 19.2 ],[38.88 38.88 46.88 38.88 46.88 46.88 46.88 38.88 ],[1 1 1 ]);
      | patch([27.2 38.76 30.76 19.2 27.2 ],[30.88 30.88 38.88 38.88 30.88 ],[0.931 0.946 0.973 ]);
      | patch([19.2 30.76 38.76 27.2 19.2 ],[22.88 22.88 30.88 30.88 22.88 ],[1 1 1 ]);
      | patch([27.2 54.76 46.76 38.76 30.76 19.2 27.2 ],[14.88 14.88 22.88 14.88 22.88 22.88 14.88 ],[0.931 0.946 0.973 ]);
      | fprintf('','COMMENT: end icon graphics');
      | fprintf('','COMMENT: begin icon text');
      | fprintf('','COMMENT: end icon text');
  "Convolutional Encoder v6_0 " : S-Function  LoadFcn=xlBlockLoadCallback(gcbh);  FunctionName=sysgen  Parameters=ptable_  EnableBusSupport=off  mask(Xilinx Convolutional Encoder Block){clength=3, conv_codes=[7 5 6], rst_sgadvanced=, rst=off, en_sgadvanced=, en=off, dbl_ovrd_sgadvanced=, dbl_ovrd=off, use_rpm_sgadvanced=, use_rpm=off, xl_use_area_sgadvanced=, xl_use_area=off, xl_area=[0,0,0,0,0,0,0], version=6, has_advanced_control=0, sggui_pos=-1,-1,-1,-1, block_type=convolutional_encoder_v6_0, block_version=, sg_icon_stat=75,60,-1,-1,white,blue,0,07734,right,,[ ],[ ], sg_mask_display=|, sg_list_contents=, sg_blockgui_xml=}
      mask sg_mask_display=|
      | fprintf('','COMMENT: begin icon graphics');
      | patch([0 75 75 0 0 ],[0 0 60 60 0 ],[0.77 0.82 0.91 ]);
      | plot([0 75 75 0 0 ],[0 0 60 60 0 ]);
      | patch([19.2 30.76 38.76 46.76 54.76 38.76 27.2 19.2 ],[38.88 38.88 46.88 38.88 46.88 46.88 46.88 38.88 ],[1 1 1 ]);
      | patch([27.2 38.76 30.76 19.2 27.2 ],[30.88 30.88 38.88 38.88 30.88 ],[0.931 0.946 0.973 ]);
      | patch([19.2 30.76 38.76 27.2 19.2 ],[22.88 22.88 30.88 30.88 22.88 ],[1 1 1 ]);
      | patch([27.2 54.76 46.76 38.76 30.76 19.2 27.2 ],[14.88 14.88 22.88 14.88 22.88 22.88 14.88 ],[0.931 0.946 0.973 ]);
      | fprintf('','COMMENT: end icon graphics');
      | fprintf('','COMMENT: begin icon text');
      | fprintf('','COMMENT: end icon text');
      mask prompts: clength "Constraint length"; conv_codes "Convolution code array (octal)"; rst_sgadvanced ""; rst "Provide synchronous reset port"; en_sgadvanced ""; en "Provide enable port"; dbl_ovrd_sgadvanced ""; dbl_ovrd "Override with doubles"; use_rpm_sgadvanced ""; use_rpm "Use core placement information"; xl_use_area_sgadvanced ""; xl_use_area "Define FPGA area for resource estimation"; xl_area "FPGA area [slices, FFs, BRAMs, LUTs, IOBs, emb. mults, TBUFs]"; version ""; has_advanced_control ""; sggui_pos ""; block_type ""; block_version ""; sg_icon_stat ""; sg_mask_display ""; sg_list_contents ""; sg_blockgui_xml ""
      mask help: Xilinx Convolutional Encoder
      mask init:
      | try
      |   tmp_gcb = gcb;
      |   tmp_gcbh = gcbh;
      |   if (strcmp('SysGenIndex',get_param(bdroot(tmp_gcbh),'tag')) && ~isempty(regexp(bdroot(tmp_gcb), '^xbs', 'once')))
      |     return;
      |   end;
      |   xlMungeMaskParams;
      |   block_config = 'sysgen_blockset:Removed_config';
      | 
      |   block_type='convolutional_encoder_v6_0';
      | nport = get_param(gcbh, 'ports');
      | nin = nport(1);
      | nout = nport(2);
      | 
      |   serialized_declarations = '{''clength''=>''Int'',''conv_codes''=>''IntVector'',''en''=>''Int'',''rst''=>''Int'',''use_rpm''=>''Int'',''version''=>''Int'',''block_type''=>''String'',''nin''=>''Double'',''nout''=>''Double''}';
      |   ptable_ = xlblockprep(get_param(tmp_gcb, 'MaskWSVariables'));
      |   try
      |     xlBlockMoveCallback(tmp_gcbh);
      |   catch 
      |      clear global xl_updateicon_recursion_guard;
      |   end;
      | catch
      |   global dbgsysgen;
      |   if(~isempty(dbgsysgen) && dbgsysgen)
      |     e = regexprep(lasterr, '\n', '\nError: ');
      |     disp(['Error: While running MaskInit code on block ' tmp_gcb ': ' e]);
      |     error(e);
      |   end
      | end
      settings: CopyFcn=xlBlockMoveCallback(gcbh);  DeleteFcn=xlDestroyGui(gcbh);  ModelCloseFcn=xlDestroyGui(gcbh);  PreSaveFcn=xlBlockPreSaveCallback(gcbh);  PostSaveFcn=xlBlockPostSaveCallback(gcbh);  DestroyFcn=xlDestroyGui(gcbh);  OpenFcn=xlOpenGui(gcbh, 'convencoderv6_gui.xml', @xlremovedenablement, -1)  CloseFcn=xlDestroyGui(gcbh);  MoveFcn=xlBlockMoveCallback(gcbh);
      mask Help: eval('');xlDoc('-book','sysgen','-topic','Convolutional_Encoder_v6_0');
      mask Display:
      | fprintf('','COMMENT: begin icon graphics');
      | patch([0 75 75 0 0 ],[0 0 60 60 0 ],[0.77 0.82 0.91 ]);
      | plot([0 75 75 0 0 ],[0 0 60 60 0 ]);
      | patch([19.2 30.76 38.76 46.76 54.76 38.76 27.2 19.2 ],[38.88 38.88 46.88 38.88 46.88 46.88 46.88 38.88 ],[1 1 1 ]);
      | patch([27.2 38.76 30.76 19.2 27.2 ],[30.88 30.88 38.88 38.88 30.88 ],[0.931 0.946 0.973 ]);
      | patch([19.2 30.76 38.76 27.2 19.2 ],[22.88 22.88 30.88 30.88 22.88 ],[1 1 1 ]);
      | patch([27.2 54.76 46.76 38.76 30.76 19.2 27.2 ],[14.88 14.88 22.88 14.88 22.88 22.88 14.88 ],[0.931 0.946 0.973 ]);
      | fprintf('','COMMENT: end icon graphics');
      | fprintf('','COMMENT: begin icon text');
      | fprintf('','COMMENT: end icon text');
  "Convolutional Encoder v6_1 " : S-Function  LoadFcn=xlBlockLoadCallback(gcbh);  FunctionName=sysgen  Parameters=ptable_  EnableBusSupport=off  mask(Xilinx Convolutional Encoder Block){clength=3, conv_codes=[7 5 6], rst_sgadvanced=, rst=off, en_sgadvanced=, en=off, dbl_ovrd_sgadvanced=, dbl_ovrd=off, use_rpm_sgadvanced=, use_rpm=off, xl_use_area_sgadvanced=, xl_use_area=off, xl_area=[0,0,0,0,0,0,0], version=61, has_advanced_control=0, sggui_pos=-1,-1,-1,-1, block_type=convolutional_encoder_v6_1, block_version=, sg_icon_stat=75,61,2,4,white,blue,0,6b56a969,right,,[ ],[ ], sg_mask_display=|, sg_list_contents=, sg_blockgui_xml=}
      mask sg_mask_display=|
      | fprintf('','COMMENT: begin icon graphics');
      | patch([0 75 75 0 0 ],[0 0 61 61 0 ],[0.77 0.82 0.91 ]);
      | plot([0 75 75 0 0 ],[0 0 61 61 0 ]);
      | patch([19.2 30.76 38.76 46.76 54.76 38.76 27.2 19.2 ],[38.88 38.88 46.88 38.88 46.88 46.88 46.88 38.88 ],[1 1 1 ]);
      | patch([27.2 38.76 30.76 19.2 27.2 ],[30.88 30.88 38.88 38.88 30.88 ],[0.931 0.946 0.973 ]);
      | patch([19.2 30.76 38.76 27.2 19.2 ],[22.88 22.88 30.88 30.88 22.88 ],[1 1 1 ]);
      | patch([27.2 54.76 46.76 38.76 30.76 19.2 27.2 ],[14.88 14.88 22.88 14.88 22.88 22.88 14.88 ],[0.931 0.946 0.973 ]);
      | fprintf('','COMMENT: end icon graphics');
      | fprintf('','COMMENT: begin icon text');
      | color('black');port_label('input',1,'din');
      | color('black');port_label('input',2,'vin');
      | color('black');port_label('output',1,'dout0');
      | color('black');port_label('output',2,'dout1');
      | color('black');port_label('output',3,'dout2');
      | color('black');port_label('output',4,'vout');
      | fprintf('','COMMENT: end icon text');
      mask prompts: clength "Constraint length"; conv_codes "Convolution code array (octal)"; rst_sgadvanced ""; rst "Provide synchronous reset port"; en_sgadvanced ""; en "Provide enable port"; dbl_ovrd_sgadvanced ""; dbl_ovrd "Override with doubles"; use_rpm_sgadvanced ""; use_rpm "Use core placement information"; xl_use_area_sgadvanced ""; xl_use_area "Define FPGA area for resource estimation"; xl_area "FPGA area [slices, FFs, BRAMs, LUTs, IOBs, emb. mults, TBUFs]"; version ""; has_advanced_control ""; sggui_pos ""; block_type ""; block_version ""; sg_icon_stat ""; sg_mask_display ""; sg_list_contents ""; sg_blockgui_xml ""
      mask help: Xilinx Convolutional Encoder
      mask init:
      | try
      |   tmp_gcb = gcb;
      |   tmp_gcbh = gcbh;
      |   if (strcmp('SysGenIndex',get_param(bdroot(tmp_gcbh),'tag')) && ~isempty(regexp(bdroot(tmp_gcb), '^xbs', 'once')))
      |     return;
      |   end;
      |   xlMungeMaskParams;
      |   block_config = 'sysgen_blockset:ConvEncoder_config';
      | 
      |   block_type='convolutional_encoder_v6_1';
      | 
      |   serialized_declarations = '{''clength''=>''Int'',''conv_codes''=>''IntVector'',''en''=>''Int'',''rst''=>''Int'',''use_rpm''=>''Int'',''version''=>''Int'',''block_type''=>''String''}';
      |   ptable_ = xlblockprep(get_param(tmp_gcb, 'MaskWSVariables'));
      |   try
      |     xlBlockMoveCallback(tmp_gcbh);
      |   catch 
      |      clear global xl_updateicon_recursion_guard;
      |   end;
      | catch
      |   global dbgsysgen;
      |   if(~isempty(dbgsysgen) && dbgsysgen)
      |     e = regexprep(lasterr, '\n', '\nError: ');
      |     disp(['Error: While running MaskInit code on block ' tmp_gcb ': ' e]);
      |     error(e);
      |   end
      | end
      settings: CopyFcn=xlBlockMoveCallback(gcbh);  DeleteFcn=xlDestroyGui(gcbh);  ModelCloseFcn=xlDestroyGui(gcbh);  PreSaveFcn=xlBlockPreSaveCallback(gcbh);  PostSaveFcn=xlBlockPostSaveCallback(gcbh);  DestroyFcn=xlDestroyGui(gcbh);  OpenFcn=xlOpenGui(gcbh, 'convencoderv61_gui.xml', @xlmagicenablement, -1)  CloseFcn=xlDestroyGui(gcbh);  MoveFcn=xlBlockMoveCallback(gcbh);
      mask Help: eval('');xlDoc('-book','sysgen','-topic','Convolutional_Encoder_v6_1');
      mask Display:
      | fprintf('','COMMENT: begin icon graphics');
      | patch([0 75 75 0 0 ],[0 0 61 61 0 ],[0.77 0.82 0.91 ]);
      | plot([0 75 75 0 0 ],[0 0 61 61 0 ]);
      | patch([19.2 30.76 38.76 46.76 54.76 38.76 27.2 19.2 ],[38.88 38.88 46.88 38.88 46.88 46.88 46.88 38.88 ],[1 1 1 ]);
      | patch([27.2 38.76 30.76 19.2 27.2 ],[30.88 30.88 38.88 38.88 30.88 ],[0.931 0.946 0.973 ]);
      | patch([19.2 30.76 38.76 27.2 19.2 ],[22.88 22.88 30.88 30.88 22.88 ],[1 1 1 ]);
      | patch([27.2 54.76 46.76 38.76 30.76 19.2 27.2 ],[14.88 14.88 22.88 14.88 22.88 22.88 14.88 ],[0.931 0.946 0.973 ]);
      | fprintf('','COMMENT: end icon graphics');
      | fprintf('','COMMENT: begin icon text');
      | color('black');port_label('input',1,'din');
      | color('black');port_label('input',2,'vin');
      | color('black');port_label('output',1,'dout0');
      | color('black');port_label('output',2,'dout1');
      | color('black');port_label('output',3,'dout2');
      | color('black');port_label('output',4,'vout');
      | fprintf('','COMMENT: end icon text');
  Counter : S-Function  LoadFcn=xlBlockLoadCallback(gcbh);  FunctionName=sysgen  Parameters=ptable_  EnableBusSupport=off  mask(Xilinx Counter Block){infoedit=Hardware notes: Free running counters are the least expensive in hardware.  A count limited counter is implemented by combining a counter with a comparator., cnt_type_sgadvanced=, cnt_type=Free Running, cnt_to=Inf, operation_sgadvanced=, operation=Up, start_count=0, cnt_by_val=1, arith_type_sgadvanced=, arith_type=Unsigned, n_bits=8, bin_pt=0, load_pin_sgadvanced=, load_pin=off, rst_sgadvanced=, rst=off, en_sgadvanced=, en=off, explicit_period_sgadvanced=, explicit_period=on, period=1, dbl_ovrd_sgadvanced=, dbl_ovrd=off, use_behavioral_HDL_sgadvanced=, use_behavioral_HDL=off, implementation_sgadvanced=, implementation=Fabric, xl_use_area_sgadvanced=, xl_use_area=off, xl_area=[0,0,0,0,0,0,0], use_rpm=, xlcconfig=, has_advanced_control=0, sggui_pos=-1,-1,-1,-1, block_type=counter, block_version=, sg_icon_stat=60,60,0,1,white,blue,0,7ac47ef5,right,,[ ],[ ], sg_mask_display=|, sg_list_contents=, sg_blockgui_xml=}
      mask sg_mask_display=|
      | fprintf('','COMMENT: begin icon graphics');
      | patch([0 60 60 0 0 ],[0 0 60 60 0 ],[0.77 0.82 0.91 ]);
      | plot([0 60 60 0 0 ],[0 0 60 60 0 ]);
      | patch([12.2 23.76 31.76 39.76 47.76 31.76 20.2 12.2 ],[38.88 38.88 46.88 38.88 46.88 46.88 46.88 38.88 ],[1 1 1 ]);
      | patch([20.2 31.76 23.76 12.2 20.2 ],[30.88 30.88 38.88 38.88 30.88 ],[0.931 0.946 0.973 ]);
      | patch([12.2 23.76 31.76 20.2 12.2 ],[22.88 22.88 30.88 30.88 22.88 ],[1 1 1 ]);
      | patch([20.2 47.76 39.76 31.76 23.76 12.2 20.2 ],[14.88 14.88 22.88 14.88 22.88 22.88 14.88 ],[0.931 0.946 0.973 ]);
      | fprintf('','COMMENT: end icon graphics');
      | fprintf('','COMMENT: begin icon text');
      |
      | color('black');disp('{\fontsize{14}\bf++}','texmode','on');
      | fprintf('','COMMENT: end icon text');
      mask prompts: infoedit ""; cnt_type_sgadvanced ""; cnt_type "Counter type"; cnt_to "Count to value"; operation_sgadvanced ""; operation "Count direction"; start_count "Initial value"; cnt_by_val "Step"; arith_type_sgadvanced ""; arith_type "Output type"; n_bits "Number of bits"; bin_pt "Binary point"; load_pin_sgadvanced ""; load_pin "Provide load port"; rst_sgadvanced ""; rst "Provide synchronous reset port"; en_sgadvanced ""; en "Provide enable port"; explicit_period_sgadvanced ""; explicit_period "Sample period source"; period "Explicit period"; dbl_ovrd_sgadvanced ""; dbl_ovrd "Override with doubles"; use_behavioral_HDL_sgadvanced ""; use_behavioral_HDL "Use behavioral HDL (otherwise use core)"; implementation_sgadvanced ""; implementation "Implement using"; xl_use_area_sgadvanced ""; xl_use_area "Define FPGA area for resource estimation"; xl_area "FPGA area [slices, FFs, BRAMs, LUTs, IOBs, emb. mults, TBUFs]"; use_rpm ""; xlcconfig ""; has_advanced_control ""; sggui_pos ""; block_type ""; block_version ""; sg_icon_stat ""; sg_mask_display ""; sg_list_contents ""; sg_blockgui_xml ""
      mask help: Hardware notes: Free running counters are the least expensive in hardware. A count limited counter is implemented by combining a counter with a comparator.
      mask init:
      | try
      |   tmp_gcb = gcb;
      |   tmp_gcbh = gcbh;
      |   if (strcmp('SysGenIndex',get_param(bdroot(tmp_gcbh),'tag')) && ~isempty(regexp(bdroot(tmp_gcb), '^xbs', 'once')))
      |     return;
      |   end;
      |   xlMungeMaskParams;
      |   block_config = 'sysgen_blockset:Counter_config';
      | 
      |   block_type='counter';
      | 
      |   serialized_declarations = '{''arith_type''=>''Int'',''bin_pt''=>''Int'',''cnt_by_val''=>''Double'',''cnt_to''=>''Double'',''cnt_type''=>''Int'',''en''=>''Int'',''explicit_period''=>''Int'',''implementation''=>''String'',''load_pin''=>''Int'',''n_bits''=>''Int'',''operation''=>''Int'',''period''=>''Double'',''rst''=>''Int'',''start_count''=>''Double'',''use_behavioral_HDL''=>''Int'',''use_rpm''=>''String'',''xlcconfig''=>''String'',''block_type''=>''String''}';
      |   ptable_ = xlblockprep(get_param(tmp_gcb, 'MaskWSVariables'));
      |   try
      |     xlBlockMoveCallback(tmp_gcbh);
      |   catch 
      |      clear global xl_updateicon_recursion_guard;
      |   end;
      | catch
      |   global dbgsysgen;
      |   if(~isempty(dbgsysgen) && dbgsysgen)
      |     e = regexprep(lasterr, '\n', '\nError: ');
      |     disp(['Error: While running MaskInit code on block ' tmp_gcb ': ' e]);
      |     error(e);
      |   end
      | end
      settings: CopyFcn=xlBlockMoveCallback(gcbh);  DeleteFcn=xlDestroyGui(gcbh);  ModelCloseFcn=xlDestroyGui(gcbh);  PreSaveFcn=xlBlockPreSaveCallback(gcbh);  PostSaveFcn=xlBlockPostSaveCallback(gcbh);  DestroyFcn=xlDestroyGui(gcbh);  OpenFcn=xlOpenGui(gcbh, 'counter_gui.xml', @counterenablement, -1)  CloseFcn=xlDestroyGui(gcbh);  MoveFcn=xlBlockMoveCallback(gcbh);
      mask Help: eval('');xlDoc('-book','sysgen','-topic','Counter');
      mask StyleString: edit,edit,popup(Free Running|Count Limited),edit,edit,popup(Up|Down|Up/Down),edit,edit,edit,popup(Signed  (2's comp)|Unsigned),edit,edit,edit,checkbox,edit,checkbox,edit,checkbox,edit,popup(on|off),edit,edit,checkbox,edit,checkbox,edit,popup(Fabric|DSP48),edit,checkbox,edit,edit,edit,edit,edit,edit,edit,edit,edit,edit,edit
      mask Display:
      | fprintf('','COMMENT: begin icon graphics');
      | patch([0 60 60 0 0 ],[0 0 60 60 0 ],[0.77 0.82 0.91 ]);
      | plot([0 60 60 0 0 ],[0 0 60 60 0 ]);
      | patch([12.2 23.76 31.76 39.76 47.76 31.76 20.2 12.2 ],[38.88 38.88 46.88 38.88 46.88 46.88 46.88 38.88 ],[1 1 1 ]);
      | patch([20.2 31.76 23.76 12.2 20.2 ],[30.88 30.88 38.88 38.88 30.88 ],[0.931 0.946 0.973 ]);
      | patch([12.2 23.76 31.76 20.2 12.2 ],[22.88 22.88 30.88 30.88 22.88 ],[1 1 1 ]);
      | patch([20.2 47.76 39.76 31.76 23.76 12.2 20.2 ],[14.88 14.88 22.88 14.88 22.88 22.88 14.88 ],[0.931 0.946 0.973 ]);
      | fprintf('','COMMENT: end icon graphics');
      | fprintf('','COMMENT: begin icon text');
      | 
      | color('black');disp('{\fontsize{14}\bf++}','texmode','on');
      | fprintf('','COMMENT: end icon text');
  "DAFIR v9_0 " : S-Function  LoadFcn=xlBlockLoadCallback(gcbh);  FunctionName=sysgen  Parameters=ptable_  EnableBusSupport=off  mask(Xilinx Finite Impulse Response Filter Block){infoedit=Hardware notes: Implemented using distributed arithmetic (DA).  The hardware over sampling rate determines the degree of parallelism.  A rate of one produces a fully parallel DA filter.  A rate of n (resp., n+1) for an n-bit input signal produces a fully serial implementation for a non-symmetric (resp., symmetric) impulse response.  Intermediate values produce implementations with intermediate levels of parallelism., coef=[1 -1], structure_sgadvanced=, structure=Inferred from Coefficients, coef_n_bits=16, coef_bin_pt=14, over_sample=1, reload_sgadvanced=, reload=off, valids_sgadvanced=, valids=off, rst_sgadvanced=, rst=off, latency=1, num_channels_sgadvanced=, num_channels=1, serial_input_sgadvanced=, serial_input=off, polyphase_behavior_sgadvanced=, polyphase_behavior=Single Rate:  sample in - sample out, dbl_ovrd_sgadvanced=, dbl_ovrd=off, xl_use_area_sgadvanced=, xl_use_area=off, xl_area=[0,0,0,0,0,0,0], explicit_period=off, period=1, use_isim=0, has_advanced_control=0, sggui_pos=-1,-1,-1,-1, block_type=fir, block_version=, sg_icon_stat=60,62,1,1,white,blue,0,292f8831,right,,[ ],[ ], sg_mask_display=|, sg_list_contents=, sg_blockgui_xml=}
      mask sg_mask_display=|
      | fprintf('','COMMENT: begin icon graphics');
      | patch([0 60 60 0 0 ],[0 0 62 62 0 ],[0.77 0.82 0.91 ]);
      | plot([0 60 60 0 0 ],[0 0 62 62 0 ]);
      | patch([12.2 23.76 31.76 39.76 47.76 31.76 20.2 12.2 ],[39.88 39.88 47.88 39.88 47.88 47.88 47.88 39.88 ],[1 1 1 ]);
      | patch([20.2 31.76 23.76 12.2 20.2 ],[31.88 31.88 39.88 39.88 31.88 ],[0.931 0.946 0.973 ]);
      | patch([12.2 23.76 31.76 20.2 12.2 ],[23.88 23.88 31.88 31.88 23.88 ],[1 1 1 ]);
      | patch([20.2 47.76 39.76 31.76 23.76 12.2 20.2 ],[15.88 15.88 23.88 15.88 23.88 23.88 15.88 ],[0.931 0.946 0.973 ]);
      | fprintf('','COMMENT: end icon graphics');
      | fprintf('','COMMENT: begin icon text');
      | color('black');port_label('input',1,'x0');
      | color('black');port_label('output',1,'y0');
      | color('black');disp('2 tap');
      | fprintf('','COMMENT: end icon text');
      mask prompts: infoedit ""; coef "Coefficients"; structure_sgadvanced ""; coef_n_bits "Number of bits (always signed)"; coef_bin_pt "Binary point"; over_sample "Hardware over-sampling rate"; reload_sgadvanced ""; reload "Provide coefficient reload ports"; valids_sgadvanced ""; valids "Provide valid ports"; rst_sgadvanced ""; rst "Provide reset port"; num_channels_sgadvanced ""; num_channels "Number of channels"; serial_input_sgadvanced ""; serial_input "Serial input"; polyphase_behavior_sgadvanced ""; polyphase_behavior "Polyphase behavior"; dbl_ovrd_sgadvanced ""; dbl_ovrd "Override with doubles"; xl_use_area_sgadvanced ""; xl_use_area "Define FPGA area for resource estimation"; xl_area "FPGA area [slices, FFs, BRAMs, LUTs, IOBs, emb. mults, TBUFs]"; explicit_period ""; period ""; use_isim ""; has_advanced_control ""; sggui_pos ""; block_type ""; block_version ""; sg_icon_stat ""; sg_mask_display ""; sg_list_contents ""; sg_blockgui_xml ""
      mask help: Hardware notes: Implemented using distributed arithmetic (DA). The hardware over sampling rate determines the degree of parallelism. A rate of one produces a fully parallel DA filter. A rate of n (resp., n+1) for an n-bit input signal produces a fully serial implementation for a non-symmetric (resp., symmetric) impulse response. Intermediate values produce implementations with intermediate levels of parallelism.
      mask init:
      | try
      |   tmp_gcb = gcb;
      |   tmp_gcbh = gcbh;
      |   if (strcmp('SysGenIndex',get_param(bdroot(tmp_gcbh),'tag')) && ~isempty(regexp(bdroot(tmp_gcb), '^xbs', 'once')))
      |     return;
      |   end;
      |   xlMungeMaskParams;
      |   block_config = 'sysgen_blockset:DAFIR_config';
      | 
      |   block_type='fir';
      | 
      |   serialized_declarations = '{''coef''=>''DoubleVector'',''coef_bin_pt''=>''Int'',''coef_n_bits''=>''Int'',''dbl_ovrd''=>''Bool'',''latency''=>''Int'',''num_channels''=>''Int'',''over_sample''=>''Int'',''polyphase_behavior''=>''Int'',''reload''=>''Bool'',''rst''=>''Bool'',''serial_input''=>''Bool'',''structure''=>''Int'',''use_isim''=>''Int'',''valids''=>''Bool'',''block_type''=>''String''}';
      |   ptable_ = xlblockprep(get_param(tmp_gcb, 'MaskWSVariables'));
      |   try
      |     xlBlockMoveCallback(tmp_gcbh);
      |   catch 
      |      clear global xl_updateicon_recursion_guard;
      |   end;
      | catch
      |   global dbgsysgen;
      |   if(~isempty(dbgsysgen) && dbgsysgen)
      |     e = regexprep(lasterr, '\n', '\nError: ');
      |     disp(['Error: While running MaskInit code on block ' tmp_gcb ': ' e]);
      |     error(e);
      |   end
      | end
      settings: CopyFcn=xlBlockMoveCallback(gcbh);  DeleteFcn=xlDestroyGui(gcbh);  ModelCloseFcn=xlDestroyGui(gcbh);  PreSaveFcn=xlBlockPreSaveCallback(gcbh);  PostSaveFcn=xlBlockPostSaveCallback(gcbh);  DestroyFcn=xlDestroyGui(gcbh);  OpenFcn=xlOpenGui(gcbh, 'dafir_gui.xml', @dafirenablement, -1)  CloseFcn=xlDestroyGui(gcbh);  MoveFcn=xlBlockMoveCallback(gcbh);
      mask Help: eval('');xlDoc('-book','sysgen','-topic','DAFIR_v9_0');
      mask StyleString: edit,edit,edit,popup(Inferred from Coefficients|None|Symmetric|Negative Symmetric|Half-Band Filter|Interpolated FIR),edit,edit,edit,edit,checkbox,edit,checkbox,edit,checkbox,edit,edit,popup(1|2|3|4|5|6|7|8),edit,checkbox,edit,popup(Decimate:  8:1 (samples in:out)|Decimate:  7:1 (samples in:out)|Decimate:  6:1 (samples in:out)|Decimate:  5:1 (samples in:out)|Decimate:  4:1 (samples in:out)|Decimate:  3:1 (samples in:out)|Decimate:  2:1 (samples in:out)|Single Rate:  sample in - sample out|Interpolate:  1:2 (samples in:out)|Interpolate:  1:3 (samples in:out)|Interpolate:  1:4 (samples in:out)|Interpolate:  1:5 (samples in:out)|Interpolate:  1:6 (samples in:out)|Interpolate:  1:7 (samples in:out)|Interpolate:  1:8 (samples in:out)),edit,checkbox,edit,checkbox,edit,edit,edit,edit,edit,edit,edit,edit,edit,edit,edit,edit
      mask Display:
      | fprintf('','COMMENT: begin icon graphics');
      | patch([0 60 60 0 0 ],[0 0 62 62 0 ],[0.77 0.82 0.91 ]);
      | plot([0 60 60 0 0 ],[0 0 62 62 0 ]);
      | patch([12.2 23.76 31.76 39.76 47.76 31.76 20.2 12.2 ],[39.88 39.88 47.88 39.88 47.88 47.88 47.88 39.88 ],[1 1 1 ]);
      | patch([20.2 31.76 23.76 12.2 20.2 ],[31.88 31.88 39.88 39.88 31.88 ],[0.931 0.946 0.973 ]);
      | patch([12.2 23.76 31.76 20.2 12.2 ],[23.88 23.88 31.88 31.88 23.88 ],[1 1 1 ]);
      | patch([20.2 47.76 39.76 31.76 23.76 12.2 20.2 ],[15.88 15.88 23.88 15.88 23.88 23.88 15.88 ],[0.931 0.946 0.973 ]);
      | fprintf('','COMMENT: end icon graphics');
      | fprintf('','COMMENT: begin icon text');
      | color('black');port_label('input',1,'x0');
      | color('black');port_label('output',1,'y0');
      | color('black');disp('2 tap');
      | fprintf('','COMMENT: end icon text');
  "DDS Compiler 2.1 " : S-Function  LoadFcn=xlBlockLoadCallback(gcbh);  FunctionName=sysgen  Parameters=ptable_  EnableBusSupport=off  mask(Xilinx DDS Compiler 2.1 Block){output_selection=Sine_and_Cosine, negative_sine=off, negative_cosine=off, channels=1, dds_clock_rate=100, spurious_free_dynamic_range=36, frequency_resolution=0.4, rst=off, en=off, rfd=off, rdy=off, channel_pin=off, explicit_period=on, period=1, phase_increment=Fixed, output_frequency1=0, output_frequency2=0, output_frequency3=0, output_frequency4=0, output_frequency5=0, output_frequency6=0, output_frequency7=0, output_frequency8=0, output_frequency9=0, output_frequency10=0, output_frequency11=0, output_frequency12=0, output_frequency13=0, output_frequency14=0, output_frequency15=0, output_frequency16=0, phase_offset=None, phase_offset_angles1=0, phase_offset_angles2=0, phase_offset_angles3=0, phase_offset_angles4=0, phase_offset_angles5=0, phase_offset_angles6=0, phase_offset_angles7=0, phase_offset_angles8=0, phase_offset_angles9=0, phase_offset_angles10=0, phase_offset_angles11=0, phase_offset_angles12=0, phase_offset_angles13=0, phase_offset_angles14=0, phase_offset_angles15=0, phase_offset_angles16=0, memory_type=Auto, optimization_goal=Auto, dsp48_use=Minimal, noise_shaping=None, latency_configuration=Auto, latency=1, accumulator_latency=One, xl_use_area=off, xl_area=[0,0,0,0,0,0,0], por_mode=false, ip_name=DDS Compiler, ip_version=2.1, dsptool_ready=true, wrapper_available=true, structural_sim=false, clock_enable=true, sclr_pin=false, port_translation_map={ 'ce' => 'en', 'sclr' => 'rst'}, has_advanced_control=0, sggui_pos=-1,-1,-1,-1, block_type=dds_compiler_v2_1, block_version=, sg_icon_stat=95,142,-1,-1,white,blue,0,07734,right,,[ ],[ ], sg_mask_display=|, sg_list_contents=, sg_blockgui_xml=}
      mask sg_mask_display=|
      | fprintf('','COMMENT: begin icon graphics');
      | patch([0 95 95 0 0 ],[0 0 142 142 0 ],[0.77 0.82 0.91 ]);
      | plot([0 95 95 0 0 ],[0 0 142 142 0 ]);
      | patch([18.075 36.86 49.86 62.86 75.86 49.86 31.075 18.075 ],[85.43 85.43 98.43 85.43 98.43 98.43 98.43 85.43 ],[1 1 1 ]);
      | patch([31.075 49.86 36.86 18.075 31.075 ],[72.43 72.43 85.43 85.43 72.43 ],[0.931 0.946 0.973 ]);
      | patch([18.075 36.86 49.86 31.075 18.075 ],[59.43 59.43 72.43 72.43 59.43 ],[1 1 1 ]);
      | patch([31.075 75.86 62.86 49.86 36.86 18.075 31.075 ],[46.43 46.43 59.43 46.43 59.43 59.43 46.43 ],[0.931 0.946 0.973 ]);
      | fprintf('','COMMENT: end icon graphics');
      | fprintf('','COMMENT: begin icon text');
      | fprintf('','COMMENT: end icon text');
      mask prompts: output_selection "Output selection"; negative_sine "Negative sine"; negative_cosine "Negative cosine"; channels "Number of channels"; dds_clock_rate "DDS clock rate (MHz)"; spurious_free_dynamic_range "Spurious free dynamic range (dB)"; frequency_resolution "Frequency resolution (Hz)"; channel_pin "channel"; explicit_period "Use explicit period"; period "Explicit period"; phase_increment ""; output_frequency1 "Frequency 1"; output_frequency2 "Frequency 2"; output_frequency3 "Frequency 3"; output_frequency4 "Frequency 4"; output_frequency5 "Frequency 5"; output_frequency6 "Frequency 6"; output_frequency7 "Frequency 7"; output_frequency8 "Frequency 8"; output_frequency9 "Frequency 9"; output_frequency10 "Frequency 10"; output_frequency11 "Frequency 11"; output_frequency12 "Frequency 12"; output_frequency13 "Frequency 13"; output_frequency14 "Frequency 14"; output_frequency15 "Frequency 15"; output_frequency16 "Frequency 16"; phase_offset ""; phase_offset_angles1 "Angle 1"; phase_offset_angles2 "Angle 2"; phase_offset_angles3 "Angle 3"; phase_offset_angles4 "Angle 4"; phase_offset_angles5 "Angle 5"; phase_offset_angles6 "Angle 6"; phase_offset_angles7 "Angle 7"; phase_offset_angles8 "Angle 8"; phase_offset_angles9 "Angle 9"; phase_offset_angles10 "Angle 10"; phase_offset_angles11 "Angle 11"; phase_offset_angles12 "Angle 12"; phase_offset_angles13 "Angle 13"; phase_offset_angles14 "Angle 14"; phase_offset_angles15 "Angle 15"; phase_offset_angles16 "Angle 16"; memory_type "Memory type"; optimization_goal "Optimization goal"; dsp48_use "Dsp48 use"; noise_shaping "Noise shaping"; latency_configuration "Latency configuration"; accumulator_latency "Accumulator latency"; xl_use_area "Define FPGA area for resource estimation"; xl_area "FPGA area [slices, FFs, BRAMs, LUTs, IOBs, emb. mults, TBUFs]"; por_mode ""; ip_name ""; ip_version ""; dsptool_ready ""; wrapper_available ""; structural_sim ""; clock_enable ""; sclr_pin ""; port_translation_map ""; has_advanced_control ""; sggui_pos ""; block_type ""; block_version ""; sg_icon_stat ""; sg_mask_display ""; sg_list_contents ""; sg_blockgui_xml ""
      mask help: Xilinx DDS Compiler 2.1
      mask init:
      | try
      |   tmp_gcb = gcb;
      |   tmp_gcbh = gcbh;
      |   if (strcmp('SysGenIndex',get_param(bdroot(tmp_gcbh),'tag')) && ~isempty(regexp(bdroot(tmp_gcb), '^xbs', 'once')))
      |     return;
      |   end;
      |   xlMungeMaskParams;
      |   block_config = 'sysgen_blockset:Removed_config';
      | 
      |   block_type='dds_compiler_v2_1';
      | nport = get_param(gcbh, 'ports');
      | nin = nport(1);
      | nout = nport(2);
      | 
      |   serialized_declarations = '{''accumulator_latency''=>''String'',''channel_pin''=>''Bool'',''channels''=>''String'',''clock_enable''=>''Bool'',''dds_clock_rate''=>''Double'',''dsp48_use''=>''String'',''dsptool_ready''=>''Bool'',''en''=>''Bool'',''explicit_period''=>''Int'',''frequency_resolution''=>''Double'',''ip_name''=>''String'',''ip_version''=>''String'',''latency''=>''String'',''latency_configuration''=>''String'',''memory_type''=>''String'',''negative_cosine''=>''Bool'',''negative_sine''=>''Bool'',''noise_shaping''=>''String'',''optimization_goal''=>''String'',''output_frequency1''=>''Double'',''output_frequency10''=>''Double'',''output_frequency11''=>''Double'',''output_frequency12''=>''Double'',''output_frequency13''=>''Double'',''output_frequency14''=>''Double'',''output_frequency15''=>''Double'',''output_frequency16''=>''Double'',''output_frequency2''=>''Double'',''output_frequency3''=>''Double'',''output_frequency4''=>''Double'',''output_frequency5''=>''Double'',''output_frequency6''=>''Double'',''output_frequency7''=>''Double'',''output_frequency8''=>''Double'',''output_frequency9''=>''Double'',''output_selection''=>''String'',''period''=>''Double'',''phase_increment''=>''String'',''phase_offset''=>''String'',''phase_offset_angles1''=>''Double'',''phase_offset_angles10''=>''Double'',''phase_offset_angles11''=>''Double'',''phase_offset_angles12''=>''Double'',''phase_offset_angles13''=>''Double'',''phase_offset_angles14''=>''Double'',''phase_offset_angles15''=>''Double'',''phase_offset_angles16''=>''Double'',''phase_offset_angles2''=>''Double'',''phase_offset_angles3''=>''Double'',''phase_offset_angles4''=>''Double'',''phase_offset_angles5''=>''Double'',''phase_offset_angles6''=>''Double'',''phase_offset_angles7''=>''Double'',''phase_offset_angles8''=>''Double'',''phase_offset_angles9''=>''Double'',''por_mode''=>''Bool'',''port_translation_map''=>''String'',''rdy''=>''Bool'',''rfd''=>''Bool'',''rst''=>''Bool'',''sclr_pin''=>''Bool'',''spurious_free_dynamic_range''=>''Double'',''structural_sim''=>''Bool'',''wrapper_available''=>''Bool'',''xl_use_area''=>''Bool'',''block_type''=>''String'',''nin''=>''Double'',''nout''=>''Double''}';
      |   xldds_compiler_v2_1_init();
      |   ptable_ = xlblockprep(get_param(tmp_gcb, 'MaskWSVariables'));
      |   try
      |     xlBlockMoveCallback(tmp_gcbh);
      |   catch 
      |      clear global xl_updateicon_recursion_guard;
      |   end;
      | catch
      |   global dbgsysgen;
      |   if(~isempty(dbgsysgen) && dbgsysgen)
      |     e = regexprep(lasterr, '\n', '\nError: ');
      |     disp(['Error: While running MaskInit code on block ' tmp_gcb ': ' e]);
      |     error(e);
      |   end
      | end
      settings: CopyFcn=xlBlockMoveCallback(gcbh);  DeleteFcn=xlDestroyGui(gcbh);  ModelCloseFcn=xlDestroyGui(gcbh);  PreSaveFcn=xlBlockPreSaveCallback(gcbh);  PostSaveFcn=xlBlockPostSaveCallback(gcbh);  DestroyFcn=xlDestroyGui(gcbh);  OpenFcn=xlOpenGui(gcbh, 'dds_compiler_v2_1_gui.xml', @xlremovedenablement, -1)  CloseFcn=xlDestroyGui(gcbh);  MoveFcn=xlBlockMoveCallback(gcbh);
      mask Help: eval('');xlDoc('-book','sysgen','-topic','DDS_Compiler_2_1');
      mask StyleString: popup(Sine|Cosine|Sine_and_Cosine),checkbox,checkbox,popup(1|2|3|4|5|6|7|8|9|10|11|12|13|14|15|16),edit,edit,edit,checkbox,checkbox,checkbox,checkbox,checkbox,checkbox,edit,popup(Fixed|Programmable),edit,edit,edit,edit,edit,edit,edit,edit,edit,edit,edit,edit,edit,edit,edit,edit,popup(None|Fixed|Programmable),edit,edit,edit,edit,edit,edit,edit,edit,edit,edit,edit,edit,edit,edit,edit,edit,popup(Auto|Distributed_ROM|Block_ROM),popup(Auto|Area|Speed),popup(Minimal|Maximal),popup(None|Phase_Dithering|Taylor_Series_Corrected|Auto),popup(Auto|Configurable),popup(1|2|3|4|5|6|7|8|9|10|11|12|13|14|15),popup(Zero|One),checkbox,edit,edit,edit,edit,edit,edit,edit,edit,edit,edit,edit,edit,edit,edit,edit,edit,edit,edit
      mask Display:
      | fprintf('','COMMENT: begin icon graphics');
      | patch([0 95 95 0 0 ],[0 0 142 142 0 ],[0.77 0.82 0.91 ]);
      | plot([0 95 95 0 0 ],[0 0 142 142 0 ]);
      | patch([18.075 36.86 49.86 62.86 75.86 49.86 31.075 18.075 ],[85.43 85.43 98.43 85.43 98.43 98.43 98.43 85.43 ],[1 1 1 ]);
      | patch([31.075 49.86 36.86 18.075 31.075 ],[72.43 72.43 85.43 85.43 72.43 ],[0.931 0.946 0.973 ]);
      | patch([18.075 36.86 49.86 31.075 18.075 ],[59.43 59.43 72.43 72.43 59.43 ],[1 1 1 ]);
      | patch([31.075 75.86 62.86 49.86 36.86 18.075 31.075 ],[46.43 46.43 59.43 46.43 59.43 59.43 46.43 ],[0.931 0.946 0.973 ]);
      | fprintf('','COMMENT: end icon graphics');
      | fprintf('','COMMENT: begin icon text');
      | fprintf('','COMMENT: end icon text');
  "DDS Compiler 3.0 " : S-Function  LoadFcn=xlBlockLoadCallback(gcbh);  FunctionName=sysgen  Parameters=ptable_  EnableBusSupport=off  mask(Xilinx DDS Compiler 3.0 Block){output_selection=Sine_and_Cosine, negative_sine=off, negative_cosine=off, channels=1, dds_clock_rate=100, spurious_free_dynamic_range=36, frequency_resolution=0.4, sclr_pin=off, clock_enable=off, rfd=off, rdy=off, channel_pin=off, explicit_period=on, period=1, phase_increment=Fixed, output_frequency1=0, output_frequency2=0, output_frequency3=0, output_frequency4=0, output_frequency5=0, output_frequency6=0, output_frequency7=0, output_frequency8=0, output_frequency9=0, output_frequency10=0, output_frequency11=0, output_frequency12=0, output_frequency13=0, output_frequency14=0, output_frequency15=0, output_frequency16=0, phase_offset=None, phase_offset_angles1=0, phase_offset_angles2=0, phase_offset_angles3=0, phase_offset_angles4=0, phase_offset_angles5=0, phase_offset_angles6=0, phase_offset_angles7=0, phase_offset_angles8=0, phase_offset_angles9=0, phase_offset_angles10=0, phase_offset_angles11=0, phase_offset_angles12=0, phase_offset_angles13=0, phase_offset_angles14=0, phase_offset_angles15=0, phase_offset_angles16=0, memory_type=Auto, optimization_goal=Auto, dsp48_use=Minimal, noise_shaping=None, latency_configuration=Auto, latency=1, accumulator_latency=One, xl_use_area=off, xl_area=[0,0,0,0,0,0,0], por_mode=false, ip_name=DDS Compiler, ip_version=3.0, dsptool_ready=true, wrapper_available=true, structural_sim=false, ipcore_verbose=false, port_translation_map={ 'ce' => 'en', 'sclr' => 'rst'}, has_advanced_control=0, sggui_pos=-1,-1,-1,-1, block_type=dds_compiler_v3_0, block_version=, sg_icon_stat=95,142,-1,-1,white,blue,0,07734,right,,[ ],[ ], sg_mask_display=|, sg_list_contents=, sg_blockgui_xml=}
      mask sg_mask_display=|
      | fprintf('','COMMENT: begin icon graphics');
      | patch([0 95 95 0 0 ],[0 0 142 142 0 ],[0.77 0.82 0.91 ]);
      | plot([0 95 95 0 0 ],[0 0 142 142 0 ]);
      | patch([18.075 36.86 49.86 62.86 75.86 49.86 31.075 18.075 ],[85.43 85.43 98.43 85.43 98.43 98.43 98.43 85.43 ],[1 1 1 ]);
      | patch([31.075 49.86 36.86 18.075 31.075 ],[72.43 72.43 85.43 85.43 72.43 ],[0.931 0.946 0.973 ]);
      | patch([18.075 36.86 49.86 31.075 18.075 ],[59.43 59.43 72.43 72.43 59.43 ],[1 1 1 ]);
      | patch([31.075 75.86 62.86 49.86 36.86 18.075 31.075 ],[46.43 46.43 59.43 46.43 59.43 59.43 46.43 ],[0.931 0.946 0.973 ]);
      | fprintf('','COMMENT: end icon graphics');
      | fprintf('','COMMENT: begin icon text');
      | fprintf('','COMMENT: end icon text');
      mask prompts: output_selection "Output selection"; negative_sine "Negative sine"; negative_cosine "Negative cosine"; channels "Number of channels"; dds_clock_rate "DDS clock rate (MHz)"; spurious_free_dynamic_range "Spurious free dynamic range (dB)"; frequency_resolution "Frequency resolution (Hz)"; sclr_pin "rst"; clock_enable "en"; channel_pin "channel"; explicit_period "Use explicit period"; period "Explicit period"; phase_increment ""; output_frequency1 "Frequency 1"; output_frequency2 "Frequency 2"; output_frequency3 "Frequency 3"; output_frequency4 "Frequency 4"; output_frequency5 "Frequency 5"; output_frequency6 "Frequency 6"; output_frequency7 "Frequency 7"; output_frequency8 "Frequency 8"; output_frequency9 "Frequency 9"; output_frequency10 "Frequency 10"; output_frequency11 "Frequency 11"; output_frequency12 "Frequency 12"; output_frequency13 "Frequency 13"; output_frequency14 "Frequency 14"; output_frequency15 "Frequency 15"; output_frequency16 "Frequency 16"; phase_offset ""; phase_offset_angles1 "Angle 1"; phase_offset_angles2 "Angle 2"; phase_offset_angles3 "Angle 3"; phase_offset_angles4 "Angle 4"; phase_offset_angles5 "Angle 5"; phase_offset_angles6 "Angle 6"; phase_offset_angles7 "Angle 7"; phase_offset_angles8 "Angle 8"; phase_offset_angles9 "Angle 9"; phase_offset_angles10 "Angle 10"; phase_offset_angles11 "Angle 11"; phase_offset_angles12 "Angle 12"; phase_offset_angles13 "Angle 13"; phase_offset_angles14 "Angle 14"; phase_offset_angles15 "Angle 15"; phase_offset_angles16 "Angle 16"; memory_type "Memory type"; optimization_goal "Optimization goal"; dsp48_use "Dsp48 use"; noise_shaping "Noise shaping"; latency_configuration "Latency configuration"; accumulator_latency "Accumulator latency"; xl_use_area "Define FPGA area for resource estimation"; xl_area "FPGA area [slices, FFs, BRAMs, LUTs, IOBs, emb. mults, TBUFs]"; por_mode ""; ip_name ""; ip_version ""; dsptool_ready ""; wrapper_available ""; structural_sim ""; ipcore_verbose ""; port_translation_map ""; has_advanced_control ""; sggui_pos ""; block_type ""; block_version ""; sg_icon_stat ""; sg_mask_display ""; sg_list_contents ""; sg_blockgui_xml ""
      mask help: Xilinx DDS Compiler 3.0
      mask init:
      | try
      |   tmp_gcb = gcb;
      |   tmp_gcbh = gcbh;
      |   if (strcmp('SysGenIndex',get_param(bdroot(tmp_gcbh),'tag')) && ~isempty(regexp(bdroot(tmp_gcb), '^xbs', 'once')))
      |     return;
      |   end;
      |   xlMungeMaskParams;
      |   block_config = 'sysgen_blockset:Removed_config';
      | 
      |   block_type='dds_compiler_v3_0';
      | nport = get_param(gcbh, 'ports');
      | nin = nport(1);
      | nout = nport(2);
      | 
      |   serialized_declarations = '{''accumulator_latency''=>''String'',''channel_pin''=>''Bool'',''channels''=>''String'',''clock_enable''=>''Bool'',''dds_clock_rate''=>''Double'',''dsp48_use''=>''String'',''dsptool_ready''=>''Bool'',''explicit_period''=>''Int'',''frequency_resolution''=>''Double'',''ip_name''=>''String'',''ip_version''=>''String'',''ipcore_verbose''=>''Bool'',''latency''=>''String'',''latency_configuration''=>''String'',''memory_type''=>''String'',''negative_cosine''=>''Bool'',''negative_sine''=>''Bool'',''noise_shaping''=>''String'',''optimization_goal''=>''String'',''output_frequency1''=>''Double'',''output_frequency10''=>''Double'',''output_frequency11''=>''Double'',''output_frequency12''=>''Double'',''output_frequency13''=>''Double'',''output_frequency14''=>''Double'',''output_frequency15''=>''Double'',''output_frequency16''=>''Double'',''output_frequency2''=>''Double'',''output_frequency3''=>''Double'',''output_frequency4''=>''Double'',''output_frequency5''=>''Double'',''output_frequency6''=>''Double'',''output_frequency7''=>''Double'',''output_frequency8''=>''Double'',''output_frequency9''=>''Double'',''output_selection''=>''String'',''period''=>''Double'',''phase_increment''=>''String'',''phase_offset''=>''String'',''phase_offset_angles1''=>''Double'',''phase_offset_angles10''=>''Double'',''phase_offset_angles11''=>''Double'',''phase_offset_angles12''=>''Double'',''phase_offset_angles13''=>''Double'',''phase_offset_angles14''=>''Double'',''phase_offset_angles15''=>''Double'',''phase_offset_angles16''=>''Double'',''phase_offset_angles2''=>''Double'',''phase_offset_angles3''=>''Double'',''phase_offset_angles4''=>''Double'',''phase_offset_angles5''=>''Double'',''phase_offset_angles6''=>''Double'',''phase_offset_angles7''=>''Double'',''phase_offset_angles8''=>''Double'',''phase_offset_angles9''=>''Double'',''por_mode''=>''Bool'',''port_translation_map''=>''String'',''rdy''=>''Bool'',''rfd''=>''Bool'',''sclr_pin''=>''Bool'',''spurious_free_dynamic_range''=>''Double'',''structural_sim''=>''Bool'',''wrapper_available''=>''Bool'',''xl_use_area''=>''Bool'',''block_type''=>''String'',''nin''=>''Double'',''nout''=>''Double''}';
      |   ptable_ = xlblockprep(get_param(tmp_gcb, 'MaskWSVariables'));
      |   try
      |     xlBlockMoveCallback(tmp_gcbh);
      |   catch 
      |      clear global xl_updateicon_recursion_guard;
      |   end;
      | catch
      |   global dbgsysgen;
      |   if(~isempty(dbgsysgen) && dbgsysgen)
      |     e = regexprep(lasterr, '\n', '\nError: ');
      |     disp(['Error: While running MaskInit code on block ' tmp_gcb ': ' e]);
      |     error(e);
      |   end
      | end
      settings: CopyFcn=xlBlockMoveCallback(gcbh);  DeleteFcn=xlDestroyGui(gcbh);  ModelCloseFcn=xlDestroyGui(gcbh);  PreSaveFcn=xlBlockPreSaveCallback(gcbh);  PostSaveFcn=xlBlockPostSaveCallback(gcbh);  DestroyFcn=xlDestroyGui(gcbh);  OpenFcn=xlOpenGui(gcbh, 'dds_compiler_v3_0_gui.xml', @xlremovedenablement, -1)  CloseFcn=xlDestroyGui(gcbh);  MoveFcn=xlBlockMoveCallback(gcbh);
      mask Help: eval('');xlDoc('-book','sysgen','-topic','DDS_Compiler_3_0');
      mask StyleString: popup(Sine|Cosine|Sine_and_Cosine),checkbox,checkbox,popup(1|2|3|4|5|6|7|8|9|10|11|12|13|14|15|16),edit,edit,edit,checkbox,checkbox,checkbox,checkbox,checkbox,checkbox,edit,popup(Fixed|Programmable),edit,edit,edit,edit,edit,edit,edit,edit,edit,edit,edit,edit,edit,edit,edit,edit,popup(None|Fixed|Programmable),edit,edit,edit,edit,edit,edit,edit,edit,edit,edit,edit,edit,edit,edit,edit,edit,popup(Auto|Distributed_ROM|Block_ROM),popup(Auto|Area|Speed),popup(Minimal|Maximal),popup(None|Phase_Dithering|Taylor_Series_Corrected|Auto),popup(Auto|Configurable),popup(1|2|3|4|5|6|7|8|9|10|11|12|13|14|15),popup(Zero|One),checkbox,edit,edit,edit,edit,edit,edit,edit,edit,edit,edit,edit,edit,edit,edit,edit,edit,edit
      mask Display:
      | fprintf('','COMMENT: begin icon graphics');
      | patch([0 95 95 0 0 ],[0 0 142 142 0 ],[0.77 0.82 0.91 ]);
      | plot([0 95 95 0 0 ],[0 0 142 142 0 ]);
      | patch([18.075 36.86 49.86 62.86 75.86 49.86 31.075 18.075 ],[85.43 85.43 98.43 85.43 98.43 98.43 98.43 85.43 ],[1 1 1 ]);
      | patch([31.075 49.86 36.86 18.075 31.075 ],[72.43 72.43 85.43 85.43 72.43 ],[0.931 0.946 0.973 ]);
      | patch([18.075 36.86 49.86 31.075 18.075 ],[59.43 59.43 72.43 72.43 59.43 ],[1 1 1 ]);
      | patch([31.075 75.86 62.86 49.86 36.86 18.075 31.075 ],[46.43 46.43 59.43 46.43 59.43 59.43 46.43 ],[0.931 0.946 0.973 ]);
      | fprintf('','COMMENT: end icon graphics');
      | fprintf('','COMMENT: begin icon text');
      | fprintf('','COMMENT: end icon text');
  "DDS Compiler 4.0 " : S-Function  LoadFcn=xlBlockLoadCallback(gcbh);  FunctionName=sysgen  Parameters=ptable_  EnableBusSupport=off  mask(Xilinx DDS Compiler 4.0 Block){partspresent=Phase_Generator_and_SIN_COS_LUT, dds_clock_rate=100, channels=1, parameter_entry=System_Parameters, spurious_free_dynamic_range=36, frequency_resolution=0.4, noise_shaping=None, phase_width=28, output_width=6, output_selection=Sine_and_Cosine, negative_sine=off, negative_cosine=off, amplitude_mode=Full_Range, memory_type=Auto, optimization_goal=Auto, dsp48_use=Minimal, latency_configuration=Auto, latency=1, has_phase_out=on, sclr_pin=off, clock_enable=off, rfd=off, rdy=off, channel_pin=off, explicit_period=off, period=1, phase_increment=Fixed, output_frequency1=0, output_frequency2=0, output_frequency3=0, output_frequency4=0, output_frequency5=0, output_frequency6=0, output_frequency7=0, output_frequency8=0, output_frequency9=0, output_frequency10=0, output_frequency11=0, output_frequency12=0, output_frequency13=0, output_frequency14=0, output_frequency15=0, output_frequency16=0, pinc1='0', pinc2='0', pinc3='0', pinc4='0', pinc5='0', pinc6='0', pinc7='0', pinc8='0', pinc9='0', pinc10='0', pinc11='0', pinc12='0', pinc13='0', pinc14='0', pinc15='0', pinc16='0', phase_offset=None, phase_offset_angles1=0, phase_offset_angles2=0, phase_offset_angles3=0, phase_offset_angles4=0, phase_offset_angles5=0, phase_offset_angles6=0, phase_offset_angles7=0, phase_offset_angles8=0, phase_offset_angles9=0, phase_offset_angles10=0, phase_offset_angles11=0, phase_offset_angles12=0, phase_offset_angles13=0, phase_offset_angles14=0, phase_offset_angles15=0, phase_offset_angles16=0, poff1='0', poff2='0', poff3='0', poff4='0', poff5='0', poff6='0', poff7='0', poff8='0', poff9='0', poff10='0', poff11='0', poff12='0', poff13='0', poff14='0', poff15='0', poff16='0', por_mode=false, gui_behaviour=Sysgen, ip_name=DDS Compiler, ip_version=4.0, dsptool_ready=true, wrapper_available=true, port_translation_map={ 'ce' => 'en', 'sclr' => 'rst' }, ipcore_xco_need_fpga_part=true, ipcore_fpga_part=xlipgetpartsetting(gcb, {'virtex4', 'xc4vsx35', '-10', 'ff668'}), ipcore_usecache=true, ipcore_useipmodelcache=true, ipcore_verbose=false, has_advanced_control=0, sggui_pos=-1,-1,-1,-1, block_type=dds_compiler_v4_0, block_version=, sg_icon_stat=95,142,0,3,white,blue,0,ea1a5d06,right,,[ ],[ ], sg_mask_display=|, sg_list_contents=, sg_blockgui_xml=}
      mask sg_mask_display=|
      | fprintf('','COMMENT: begin icon graphics');
      | patch([0 95 95 0 0 ],[0 0 142 142 0 ],[0.77 0.82 0.91 ]);
      | plot([0 95 95 0 0 ],[0 0 142 142 0 ]);
      | patch([18.075 36.86 49.86 62.86 75.86 49.86 31.075 18.075 ],[85.43 85.43 98.43 85.43 98.43 98.43 98.43 85.43 ],[1 1 1 ]);
      | patch([31.075 49.86 36.86 18.075 31.075 ],[72.43 72.43 85.43 85.43 72.43 ],[0.931 0.946 0.973 ]);
      | patch([18.075 36.86 49.86 31.075 18.075 ],[59.43 59.43 72.43 72.43 59.43 ],[1 1 1 ]);
      | patch([31.075 75.86 62.86 49.86 36.86 18.075 31.075 ],[46.43 46.43 59.43 46.43 59.43 59.43 46.43 ],[0.931 0.946 0.973 ]);
      | fprintf('','COMMENT: end icon graphics');
      | fprintf('','COMMENT: begin icon text');
      | color('black');port_label('output',1,'sine');
      | color('black');port_label('output',2,'cosine');
      | color('black');port_label('output',3,'phase_out');
      | fprintf('','COMMENT: end icon text');
      mask prompts: partspresent "Configuration Options"; dds_clock_rate "System Clock (Mhz)"; channels "Number of Channels"; parameter_entry "Parameter Selection"; spurious_free_dynamic_range "Spurious Free Dynamic Range (dB)"; frequency_resolution "Frequency Resolution (Hz)"; noise_shaping "Noise Shaping"; phase_width "Phase Width"; output_width "Output Width"; output_selection ""; negative_sine "Negative Sine"; negative_cosine "Negative Cosine"; amplitude_mode "Amplitude Mode"; memory_type "Memory Type"; optimization_goal "Optimization Goal"; dsp48_use "DSP48 Use"; latency_configuration ""; has_phase_out "Has phase out"; sclr_pin "rst"; clock_enable "en"; channel_pin "Channel pin"; explicit_period "Use explicit period"; period "Explicit Period"; phase_increment ""; output_frequency1 "Channel 1"; output_frequency2 "Channel 2"; output_frequency3 "Channel 3"; output_frequency4 "Channel 4"; output_frequency5 "Channel 5"; output_frequency6 "Channel 6"; output_frequency7 "Channel 7"; output_frequency8 "Channel 8"; output_frequency9 "Channel 9"; output_frequency10 "Channel 10"; output_frequency11 "Channel 11"; output_frequency12 "Channel 12"; output_frequency13 "Channel 13"; output_frequency14 "Channel 14"; output_frequency15 "Channel 15"; output_frequency16 "Channel 16"; pinc1 "Channel 1"; pinc2 "Channel 2"; pinc3 "Channel 3"; pinc4 "Channel 4"; pinc5 "Channel 5"; pinc6 "Channel 6"; pinc7 "Channel 7"; pinc8 "Channel 8"; pinc9 "Channel 9"; pinc10 "Channel 10"; pinc11 "Channel 11"; pinc12 "Channel 12"; pinc13 "Channel 13"; pinc14 "Channel 14"; pinc15 "Channel 15"; pinc16 "Channel 16"; phase_offset ""; phase_offset_angles1 "Channel 1"; phase_offset_angles2 "Channel 2"; phase_offset_angles3 "Channel 3"; phase_offset_angles4 "Channel 4"; phase_offset_angles5 "Channel 5"; phase_offset_angles6 "Channel 6"; phase_offset_angles7 "Channel 7"; phase_offset_angles8 "Channel 8"; phase_offset_angles9 "Channel 9"; phase_offset_angles10 "Channel 10"; phase_offset_angles11 "Channel 11"; phase_offset_angles12 "Channel 12"; phase_offset_angles13 "Channel 13"; phase_offset_angles14 "Channel 14"; phase_offset_angles15 "Channel 15"; phase_offset_angles16 "Channel 16"; poff1 "Channel 1"; poff2 "Channel 2"; poff3 "Channel 3"; poff4 "Channel 4"; poff5 "Channel 5"; poff6 "Channel 6"; poff7 "Channel 7"; poff8 "Channel 8"; poff9 "Channel 9"; poff10 "Channel 10"; poff11 "Channel 11"; poff12 "Channel 12"; poff13 "Channel 13"; poff14 "Channel 14"; poff15 "Channel 15"; poff16 "Channel 16"; por_mode ""; gui_behaviour ""; ip_name ""; ip_version ""; dsptool_ready ""; wrapper_available ""; port_translation_map ""; ipcore_xco_need_fpga_part ""; ipcore_fpga_part ""; ipcore_usecache ""; ipcore_useipmodelcache ""; ipcore_verbose ""; has_advanced_control ""; sggui_pos ""; block_type ""; block_version ""; sg_icon_stat ""; sg_mask_display ""; sg_list_contents ""; sg_blockgui_xml ""
      mask help: Xilinx DDS Compiler 4.0
      mask init:
      | try
      |   tmp_gcb = gcb;
      |   tmp_gcbh = gcbh;
      |   if (strcmp('SysGenIndex',get_param(bdroot(tmp_gcbh),'tag')) && ~isempty(regexp(bdroot(tmp_gcb), '^xbs', 'once')))
      |     return;
      |   end;
      |   xlMungeMaskParams;
      |   block_config = 'sysgen:coregenimport_config';
      | 
      |   block_type='dds_compiler_v4_0';
      | 
      |   serialized_declarations = '{''amplitude_mode''=>''String'',''channel_pin''=>''Bool'',''channels''=>''String'',''clock_enable''=>''Bool'',''dds_clock_rate''=>''Double'',''dsp48_use''=>''String'',''dsptool_ready''=>''Bool'',''explicit_period''=>''Bool'',''frequency_resolution''=>''Double'',''gui_behaviour''=>''String'',''has_phase_out''=>''Bool'',''ip_name''=>''String'',''ip_version''=>''String'',''ipcore_fpga_part''=>''StringVector'',''ipcore_usecache''=>''Bool'',''ipcore_useipmodelcache''=>''Bool'',''ipcore_verbose''=>''Bool'',''ipcore_xco_need_fpga_part''=>''Bool'',''latency''=>''String'',''latency_configuration''=>''String'',''memory_type''=>''String'',''negative_cosine''=>''Bool'',''negative_sine''=>''Bool'',''noise_shaping''=>''String'',''optimization_goal''=>''String'',''output_frequency1''=>''Double'',''output_frequency10''=>''Double'',''output_frequency11''=>''Double'',''output_frequency12''=>''Double'',''output_frequency13''=>''Double'',''output_frequency14''=>''Double'',''output_frequency15''=>''Double'',''output_frequency16''=>''Double'',''output_frequency2''=>''Double'',''output_frequency3''=>''Double'',''output_frequency4''=>''Double'',''output_frequency5''=>''Double'',''output_frequency6''=>''Double'',''output_frequency7''=>''Double'',''output_frequency8''=>''Double'',''output_frequency9''=>''Double'',''output_selection''=>''String'',''output_width''=>''Int'',''parameter_entry''=>''String'',''partspresent''=>''String'',''period''=>''Double'',''phase_increment''=>''String'',''phase_offset''=>''String'',''phase_offset_angles1''=>''Double'',''phase_offset_angles10''=>''Double'',''phase_offset_angles11''=>''Double'',''phase_offset_angles12''=>''Double'',''phase_offset_angles13''=>''Double'',''phase_offset_angles14''=>''Double'',''phase_offset_angles15''=>''Double'',''phase_offset_angles16''=>''Double'',''phase_offset_angles2''=>''Double'',''phase_offset_angles3''=>''Double'',''phase_offset_angles4''=>''Double'',''phase_offset_angles5''=>''Double'',''phase_offset_angles6''=>''Double'',''phase_offset_angles7''=>''Double'',''phase_offset_angles8''=>''Double'',''phase_offset_angles9''=>''Double'',''phase_width''=>''Int'',''pinc1''=>''String'',''pinc10''=>''String'',''pinc11''=>''String'',''pinc12''=>''String'',''pinc13''=>''String'',''pinc14''=>''String'',''pinc15''=>''String'',''pinc16''=>''String'',''pinc2''=>''String'',''pinc3''=>''String'',''pinc4''=>''String'',''pinc5''=>''String'',''pinc6''=>''String'',''pinc7''=>''String'',''pinc8''=>''String'',''pinc9''=>''String'',''poff1''=>''String'',''poff10''=>''String'',''poff11''=>''String'',''poff12''=>''String'',''poff13''=>''String'',''poff14''=>''String'',''poff15''=>''String'',''poff16''=>''String'',''poff2''=>''String'',''poff3''=>''String'',''poff4''=>''String'',''poff5''=>''String'',''poff6''=>''String'',''poff7''=>''String'',''poff8''=>''String'',''poff9''=>''String'',''por_mode''=>''Bool'',''port_translation_map''=>''String'',''rdy''=>''Bool'',''rfd''=>''Bool'',''sclr_pin''=>''Bool'',''spurious_free_dynamic_range''=>''Double'',''wrapper_available''=>''Bool'',''block_type''=>''String''}';
      |   ptable_ = xlblockprep(get_param(tmp_gcb, 'MaskWSVariables'));
      |   try
      |     xlBlockMoveCallback(tmp_gcbh);
      |   catch 
      |      clear global xl_updateicon_recursion_guard;
      |   end;
      | catch
      |   global dbgsysgen;
      |   if(~isempty(dbgsysgen) && dbgsysgen)
      |     e = regexprep(lasterr, '\n', '\nError: ');
      |     disp(['Error: While running MaskInit code on block ' tmp_gcb ': ' e]);
      |     error(e);
      |   end
      | end
      settings: CopyFcn=xlBlockMoveCallback(gcbh);  DeleteFcn=xlDestroyGui(gcbh);  ModelCloseFcn=xlDestroyGui(gcbh);  PreSaveFcn=xlBlockPreSaveCallback(gcbh);  PostSaveFcn=xlBlockPostSaveCallback(gcbh);  DestroyFcn=xlDestroyGui(gcbh);  OpenFcn=xlOpenGui(gcbh, 'dds_compiler_v4_0_gui.xml', @xlipmagiccallback, @xlipmagicaction)  CloseFcn=xlDestroyGui(gcbh);  MoveFcn=xlBlockMoveCallback(gcbh);
      mask Help: eval('');xlDoc('-book','sysgen','-topic','DDS_Compiler_4_0');
      mask StyleString: popup(Phase_Generator_and_SIN_COS_LUT|Phase_Generator_only|SIN_COS_LUT_only),edit,popup(1|2|3|4|5|6|7|8|9|10|11|12|13|14|15|16),popup(System_Parameters|Hardware_Parameters),edit,edit,popup(None|Phase_Dithering|Taylor_Series_Corrected|Auto),edit,edit,popup(Sine_and_Cosine|Sine|Cosine),checkbox,checkbox,popup(Full_Range|Unit_Circle),popup(Auto|Distributed_ROM|Block_ROM),popup(Auto|Area|Speed),popup(Minimal|Maximal),popup(Auto|Configurable),popup(1|2|3|4|5|6|7|8|9|10|11|12|13|14|15),checkbox,checkbox,checkbox,checkbox,checkbox,checkbox,checkbox,edit,popup(Fixed|Programmable|Streaming),edit,edit,edit,edit,edit,edit,edit,edit,edit,edit,edit,edit,edit,edit,edit,edit,edit,edit,edit,edit,edit,edit,edit,edit,edit,edit,edit,edit,edit,edit,edit,edit,popup(None|Fixed|Programmable|Streaming),edit,edit,edit,edit,edit,edit,edit,edit,edit,edit,edit,edit,edit,edit,edit,edit,edit,edit,edit,edit,edit,edit,edit,edit,edit,edit,edit,edit,edit,edit,edit,edit,edit,edit,edit,edit,edit,edit,edit,edit,edit,edit,edit,edit,edit,edit,edit,edit,edit,edit,edit,edit
      mask Display:
      | fprintf('','COMMENT: begin icon graphics');
      | patch([0 95 95 0 0 ],[0 0 142 142 0 ],[0.77 0.82 0.91 ]);
      | plot([0 95 95 0 0 ],[0 0 142 142 0 ]);
      | patch([18.075 36.86 49.86 62.86 75.86 49.86 31.075 18.075 ],[85.43 85.43 98.43 85.43 98.43 98.43 98.43 85.43 ],[1 1 1 ]);
      | patch([31.075 49.86 36.86 18.075 31.075 ],[72.43 72.43 85.43 85.43 72.43 ],[0.931 0.946 0.973 ]);
      | patch([18.075 36.86 49.86 31.075 18.075 ],[59.43 59.43 72.43 72.43 59.43 ],[1 1 1 ]);
      | patch([31.075 75.86 62.86 49.86 36.86 18.075 31.075 ],[46.43 46.43 59.43 46.43 59.43 59.43 46.43 ],[0.931 0.946 0.973 ]);
      | fprintf('','COMMENT: end icon graphics');
      | fprintf('','COMMENT: begin icon text');
      | color('black');port_label('output',1,'sine');
      | color('black');port_label('output',2,'cosine');
      | color('black');port_label('output',3,'phase_out');
      | fprintf('','COMMENT: end icon text');
  "DDS Compiler 5.0 " : S-Function  LoadFcn=xlBlockLoadCallback(gcbh);  FunctionName=sysgen  Parameters=ptable_  EnableBusSupport=off  mask(Xilinx DDS Compiler 5.0 Block){partspresent=Phase_Generator_and_SIN_COS_LUT, dds_clock_rate=100, channels=1, parameter_entry=System_Parameters, spurious_free_dynamic_range=36, frequency_resolution=0.4, noise_shaping=None, phase_width=28, output_width=6, output_selection=Sine_and_Cosine, negative_sine=off, negative_cosine=off, amplitude_mode=Full_Range, memory_type=Auto, optimization_goal=Auto, dsp48_use=Minimal, latency_configuration=Auto, latency=1, has_phase_out=on, has_aclken=off, has_aresetn=off, explicit_period=off, period=1, data_has_tlast=Not_Required, has_tready=on, s_phase_has_tuser=Not_Required, m_data_has_tuser=Not_Required, m_phase_has_tuser=Not_Required, s_phase_tuser_width=1, s_config_sync_mode=On_Vector, phase_increment=Fixed, output_frequency1=0, output_frequency2=0, output_frequency3=0, output_frequency4=0, output_frequency5=0, output_frequency6=0, output_frequency7=0, output_frequency8=0, output_frequency9=0, output_frequency10=0, output_frequency11=0, output_frequency12=0, output_frequency13=0, output_frequency14=0, output_frequency15=0, output_frequency16=0, pinc1='0', pinc2='0', pinc3='0', pinc4='0', pinc5='0', pinc6='0', pinc7='0', pinc8='0', pinc9='0', pinc10='0', pinc11='0', pinc12='0', pinc13='0', pinc14='0', pinc15='0', pinc16='0', phase_offset=None, phase_offset_angles1=0, phase_offset_angles2=0, phase_offset_angles3=0, phase_offset_angles4=0, phase_offset_angles5=0, phase_offset_angles6=0, phase_offset_angles7=0, phase_offset_angles8=0, phase_offset_angles9=0, phase_offset_angles10=0, phase_offset_angles11=0, phase_offset_angles12=0, phase_offset_angles13=0, phase_offset_angles14=0, phase_offset_angles15=0, phase_offset_angles16=0, poff1='0', poff2='0', poff3='0', poff4='0', poff5='0', poff6='0', poff7='0', poff8='0', poff9='0', poff10='0', poff11='0', poff12='0', poff13='0', poff14='0', poff15='0', poff16='0', trim_axipin_name=on, por_mode=false, gui_behaviour=Sysgen, ip_name=DDS Compiler, ip_version=5.0, dsptool_ready=true, wrapper_available=true, port_translation_map={ 'aclken' => 'en', 'aresetn' => 'rst' }, ipcore_xco_need_fpga_part=true, ipcore_fpga_part=xlipgetpartsetting(gcb, {'virtex6', 'xc6vlx75t', '-3', 'ff784'}), ipcore_usecache=true, ipcore_useipmodelcache=true, ipcore_verbose=false, has_advanced_control=0, sggui_pos=-1,-1,-1,-1, block_type=dds_compiler_v5_0, block_version=, sg_icon_stat=245,262,2,5,white,blue,0,16b2e36b,right,,[2 3 ],[2 2 2 3 3 ], sg_mask_display=|, sg_list_contents=, sg_blockgui_xml=}
      mask sg_mask_display=|
      | fprintf('','COMMENT: begin icon graphics');
      | patch([0 0 4 4 ],[240 152 152 240 ],[5.466667e-001 5.800000e-001 6.400000e-001 ]);
      | patch([0 0 4 4 ],[110 22 22 110 ],[3.233333e-001 3.400000e-001 3.700000e-001 ]);
      | patch([241 241 245 245 ],[248 114 114 248 ],[5.466667e-001 5.800000e-001 6.400000e-001 ]);
      | patch([241 241 245 245 ],[98 14 14 98 ],[3.233333e-001 3.400000e-001 3.700000e-001 ]);
      | patch([4 240 240 4 4 ],[0 0 262 262 0 ],[7.700000e-001 8.200000e-001 9.100000e-001 ]);
      | plot([4 240 240 4 4 ],[0 0 262 262 0 ]);
      |
      |
      | patch([44.125 94.7 129.7 164.7 199.7 129.7 79.125 44.125 ],[169.85 169.85 204.85 169.85 204.85 204.85 204.85 169.85 ],[1 1 1 ]);
      | patch([79.125 129.7 94.7 44.125 79.125 ],[134.85 134.85 169.85 169.85 134.85 ],[0.931 0.946 0.973 ]);
      | patch([44.125 94.7 129.7 79.125 44.125 ],[99.85 99.85 134.85 134.85 99.85 ],[1 1 1 ]);
      | patch([79.125 199.7 164.7 129.7 94.7 44.125 79.125 ],[64.85 64.85 99.85 64.85 99.85 99.85 64.85 ],[0.931 0.946 0.973 ]);
      | fprintf('','COMMENT: end icon graphics');
      | fprintf('','COMMENT: begin icon text');
      | color('black');port_label('input',1,'  data_tready  ');
      | color('black');port_label('input',2,'  phase_tready  ');
      | color('black');port_label('output',1,'  data_tvalid  ');
      | color('black');port_label('output',2,'  data_tdata_sine  ');
      | color('black');port_label('output',3,'  data_tdata_cosine  ');
      | color('black');port_label('output',4,'  phase_tvalid  ');
      | color('black');port_label('output',5,'  phase_tdata  ');
      | fprintf('','COMMENT: end icon text');
      mask prompts: partspresent "Configuration Options"; dds_clock_rate "System Clock (MHz)"; channels "Number of Channels"; parameter_entry "Parameter Selection"; spurious_free_dynamic_range "Spurious Free Dynamic Range (dB)"; frequency_resolution "Frequency Resolution (Hz)"; noise_shaping "Noise Shaping"; phase_width "Phase Width"; output_width "Output Width"; output_selection ""; negative_sine "Negative Sine"; negative_cosine "Negative Cosine"; amplitude_mode "Amplitude Mode"; memory_type "Memory Type"; optimization_goal "Optimization Goal"; dsp48_use "DSP48 Use"; latency_configuration ""; has_phase_out "Has phase out"; has_aclken "ACLKEN"; has_aresetn "ARESETn"; explicit_period "Use explicit period"; period "Explicit Period"; data_has_tlast ""; has_tready "Output TREADY"; s_phase_has_tuser "Input"; m_data_has_tuser "DATA Output"; m_phase_has_tuser "PHASE Output"; s_phase_tuser_width "User Field Width"; s_config_sync_mode "Synchronization Mode"; phase_increment ""; output_frequency1 "Channel 1"; output_frequency2 "Channel 2"; output_frequency3 "Channel 3"; output_frequency4 "Channel 4"; output_frequency5 "Channel 5"; output_frequency6 "Channel 6"; output_frequency7 "Channel 7"; output_frequency8 "Channel 8"; output_frequency9 "Channel 9"; output_frequency10 "Channel 10"; output_frequency11 "Channel 11"; output_frequency12 "Channel 12"; output_frequency13 "Channel 13"; output_frequency14 "Channel 14"; output_frequency15 "Channel 15"; output_frequency16 "Channel 16"; pinc1 "Channel 1"; pinc2 "Channel 2"; pinc3 "Channel 3"; pinc4 "Channel 4"; pinc5 "Channel 5"; pinc6 "Channel 6"; pinc7 "Channel 7"; pinc8 "Channel 8"; pinc9 "Channel 9"; pinc10 "Channel 10"; pinc11 "Channel 11"; pinc12 "Channel 12"; pinc13 "Channel 13"; pinc14 "Channel 14"; pinc15 "Channel 15"; pinc16 "Channel 16"; phase_offset ""; phase_offset_angles1 "Channel 1"; phase_offset_angles2 "Channel 2"; phase_offset_angles3 "Channel 3"; phase_offset_angles4 "Channel 4"; phase_offset_angles5 "Channel 5"; phase_offset_angles6 "Channel 6"; phase_offset_angles7 "Channel 7"; phase_offset_angles8 "Channel 8"; phase_offset_angles9 "Channel 9"; phase_offset_angles10 "Channel 10"; phase_offset_angles11 "Channel 11"; phase_offset_angles12 "Channel 12"; phase_offset_angles13 "Channel 13"; phase_offset_angles14 "Channel 14"; phase_offset_angles15 "Channel 15"; phase_offset_angles16 "Channel 16"; poff1 "Channel 1"; poff2 "Channel 2"; poff3 "Channel 3"; poff4 "Channel 4"; poff5 "Channel 5"; poff6 "Channel 6"; poff7 "Channel 7"; poff8 "Channel 8"; poff9 "Channel 9"; poff10 "Channel 10"; poff11 "Channel 11"; poff12 "Channel 12"; poff13 "Channel 13"; poff14 "Channel 14"; poff15 "Channel 15"; poff16 "Channel 16"; trim_axipin_name "Display shortened port names"; por_mode ""; gui_behaviour ""; ip_name ""; ip_version ""; dsptool_ready ""; wrapper_available ""; port_translation_map ""; ipcore_xco_need_fpga_part ""; ipcore_fpga_part ""; ipcore_usecache ""; ipcore_useipmodelcache ""; ipcore_verbose ""; has_advanced_control ""; sggui_pos ""; block_type ""; block_version ""; sg_icon_stat ""; sg_mask_display ""; sg_list_contents ""; sg_blockgui_xml ""
      mask help: Xilinx DDS Compiler 5.0
      mask init:
      | try
      |   tmp_gcb = gcb;
      |   tmp_gcbh = gcbh;
      |   if (strcmp('SysGenIndex',get_param(bdroot(tmp_gcbh),'tag')) && ~isempty(regexp(bdroot(tmp_gcb), '^xbs', 'once')))
      |     return;
      |   end;
      |   xlMungeMaskParams;
      |   block_config = 'sysgen:coregenimport_config';
      | 
      |   block_type='dds_compiler_v5_0';
      | 
      |   serialized_declarations = '{''amplitude_mode''=>''String'',''channels''=>''String'',''data_has_tlast''=>''String'',''dds_clock_rate''=>''Double'',''dsp48_use''=>''String'',''dsptool_ready''=>''Bool'',''explicit_period''=>''Bool'',''frequency_resolution''=>''Double'',''gui_behaviour''=>''String'',''has_aclken''=>''Bool'',''has_aresetn''=>''Bool'',''has_phase_out''=>''Bool'',''has_tready''=>''Bool'',''ip_name''=>''String'',''ip_version''=>''String'',''ipcore_fpga_part''=>''StringVector'',''ipcore_usecache''=>''Bool'',''ipcore_useipmodelcache''=>''Bool'',''ipcore_verbose''=>''Bool'',''ipcore_xco_need_fpga_part''=>''Bool'',''latency''=>''String'',''latency_configuration''=>''String'',''m_data_has_tuser''=>''String'',''m_phase_has_tuser''=>''String'',''memory_type''=>''String'',''negative_cosine''=>''Bool'',''negative_sine''=>''Bool'',''noise_shaping''=>''String'',''optimization_goal''=>''String'',''output_frequency1''=>''Double'',''output_frequency10''=>''Double'',''output_frequency11''=>''Double'',''output_frequency12''=>''Double'',''output_frequency13''=>''Double'',''output_frequency14''=>''Double'',''output_frequency15''=>''Double'',''output_frequency16''=>''Double'',''output_frequency2''=>''Double'',''output_frequency3''=>''Double'',''output_frequency4''=>''Double'',''output_frequency5''=>''Double'',''output_frequency6''=>''Double'',''output_frequency7''=>''Double'',''output_frequency8''=>''Double'',''output_frequency9''=>''Double'',''output_selection''=>''String'',''output_width''=>''Int'',''parameter_entry''=>''String'',''partspresent''=>''String'',''period''=>''Double'',''phase_increment''=>''String'',''phase_offset''=>''String'',''phase_offset_angles1''=>''Double'',''phase_offset_angles10''=>''Double'',''phase_offset_angles11''=>''Double'',''phase_offset_angles12''=>''Double'',''phase_offset_angles13''=>''Double'',''phase_offset_angles14''=>''Double'',''phase_offset_angles15''=>''Double'',''phase_offset_angles16''=>''Double'',''phase_offset_angles2''=>''Double'',''phase_offset_angles3''=>''Double'',''phase_offset_angles4''=>''Double'',''phase_offset_angles5''=>''Double'',''phase_offset_angles6''=>''Double'',''phase_offset_angles7''=>''Double'',''phase_offset_angles8''=>''Double'',''phase_offset_angles9''=>''Double'',''phase_width''=>''Int'',''pinc1''=>''String'',''pinc10''=>''String'',''pinc11''=>''String'',''pinc12''=>''String'',''pinc13''=>''String'',''pinc14''=>''String'',''pinc15''=>''String'',''pinc16''=>''String'',''pinc2''=>''String'',''pinc3''=>''String'',''pinc4''=>''String'',''pinc5''=>''String'',''pinc6''=>''String'',''pinc7''=>''String'',''pinc8''=>''String'',''pinc9''=>''String'',''poff1''=>''String'',''poff10''=>''String'',''poff11''=>''String'',''poff12''=>''String'',''poff13''=>''String'',''poff14''=>''String'',''poff15''=>''String'',''poff16''=>''String'',''poff2''=>''String'',''poff3''=>''String'',''poff4''=>''String'',''poff5''=>''String'',''poff6''=>''String'',''poff7''=>''String'',''poff8''=>''String'',''poff9''=>''String'',''por_mode''=>''Bool'',''port_translation_map''=>''String'',''s_config_sync_mode''=>''String'',''s_phase_has_tuser''=>''String'',''s_phase_tuser_width''=>''Int'',''spurious_free_dynamic_range''=>''Double'',''trim_axipin_name''=>''Int'',''wrapper_available''=>''Bool'',''block_type''=>''String''}';
      |   ptable_ = xlblockprep(get_param(tmp_gcb, 'MaskWSVariables'));
      |   try
      |     xlBlockMoveCallback(tmp_gcbh);
      |   catch 
      |      clear global xl_updateicon_recursion_guard;
      |   end;
      | catch
      |   global dbgsysgen;
      |   if(~isempty(dbgsysgen) && dbgsysgen)
      |     e = regexprep(lasterr, '\n', '\nError: ');
      |     disp(['Error: While running MaskInit code on block ' tmp_gcb ': ' e]);
      |     error(e);
      |   end
      | end
      settings: CopyFcn=xlBlockMoveCallback(gcbh);  DeleteFcn=xlDestroyGui(gcbh);  ModelCloseFcn=xlDestroyGui(gcbh);  PreSaveFcn=xlBlockPreSaveCallback(gcbh);  PostSaveFcn=xlBlockPostSaveCallback(gcbh);  DestroyFcn=xlDestroyGui(gcbh);  OpenFcn=xlOpenGui(gcbh, 'dds_compiler_v5_0_gui.xml', @xlipmagiccallback, @dds_compiler_5_0_action)  CloseFcn=xlDestroyGui(gcbh);  MoveFcn=xlBlockMoveCallback(gcbh);
      mask Help: eval('');xlDoc('-book','sysgen','-topic','DDS_Compiler_5_0');
      mask StyleString: popup(Phase_Generator_and_SIN_COS_LUT|Phase_Generator_only|SIN_COS_LUT_only),edit,popup(1|2|3|4|5|6|7|8|9|10|11|12|13|14|15|16),popup(System_Parameters|Hardware_Parameters),edit,edit,popup(None|Phase_Dithering|Taylor_Series_Corrected|Auto),edit,edit,popup(Sine_and_Cosine|Sine|Cosine),checkbox,checkbox,popup(Full_Range|Unit_Circle),popup(Auto|Distributed_ROM|Block_ROM),popup(Auto|Area|Speed),popup(Minimal|Maximal),popup(Auto|Configurable),popup(1|2|3|4|5|6|7|8|9|10|11|12|13|14|15),checkbox,checkbox,checkbox,checkbox,edit,popup(Not_Required|Vector_Framing|Packet_Framing|Config_Triggered),checkbox,popup(Not_Required|Chan_ID_Field|User_Field|User_and_Chan_ID_Field),popup(Not_Required|Chan_ID_Field|User_Field|User_and_Chan_ID_Field),popup(Not_Required|Chan_ID_Field|User_Field|User_and_Chan_ID_Field),edit,popup(On_Vector|On_Packet),popup(Fixed|Programmable|Streaming),edit,edit,edit,edit,edit,edit,edit,edit,edit,edit,edit,edit,edit,edit,edit,edit,edit,edit,edit,edit,edit,edit,edit,edit,edit,edit,edit,edit,edit,edit,edit,edit,popup(None|Fixed|Programmable|Streaming),edit,edit,edit,edit,edit,edit,edit,edit,edit,edit,edit,edit,edit,edit,edit,edit,edit,edit,edit,edit,edit,edit,edit,edit,edit,edit,edit,edit,edit,edit,edit,edit,checkbox,edit,edit,edit,edit,edit,edit,edit,edit,edit,edit,edit,edit,edit,edit,edit,edit,edit,edit,edit,edit
      mask Display:
      | fprintf('','COMMENT: begin icon graphics');
      | patch([0 0 4 4 ],[240 152 152 240 ],[5.466667e-001 5.800000e-001 6.400000e-001 ]);
      | patch([0 0 4 4 ],[110 22 22 110 ],[3.233333e-001 3.400000e-001 3.700000e-001 ]);
      | patch([241 241 245 245 ],[248 114 114 248 ],[5.466667e-001 5.800000e-001 6.400000e-001 ]);
      | patch([241 241 245 245 ],[98 14 14 98 ],[3.233333e-001 3.400000e-001 3.700000e-001 ]);
      | patch([4 240 240 4 4 ],[0 0 262 262 0 ],[7.700000e-001 8.200000e-001 9.100000e-001 ]);
      | plot([4 240 240 4 4 ],[0 0 262 262 0 ]);
      | 
      | 
      | patch([44.125 94.7 129.7 164.7 199.7 129.7 79.125 44.125 ],[169.85 169.85 204.85 169.85 204.85 204.85 204.85 169.85 ],[1 1 1 ]);
      | patch([79.125 129.7 94.7 44.125 79.125 ],[134.85 134.85 169.85 169.85 134.85 ],[0.931 0.946 0.973 ]);
      | patch([44.125 94.7 129.7 79.125 44.125 ],[99.85 99.85 134.85 134.85 99.85 ],[1 1 1 ]);
      | patch([79.125 199.7 164.7 129.7 94.7 44.125 79.125 ],[64.85 64.85 99.85 64.85 99.85 99.85 64.85 ],[0.931 0.946 0.973 ]);
      | fprintf('','COMMENT: end icon graphics');
      | fprintf('','COMMENT: begin icon text');
      | color('black');port_label('input',1,'  data_tready  ');
      | color('black');port_label('input',2,'  phase_tready  ');
      | color('black');port_label('output',1,'  data_tvalid  ');
      | color('black');port_label('output',2,'  data_tdata_sine  ');
      | color('black');port_label('output',3,'  data_tdata_cosine  ');
      | color('black');port_label('output',4,'  phase_tvalid  ');
      | color('black');port_label('output',5,'  phase_tdata  ');
      | fprintf('','COMMENT: end icon text');
  "DDS Compiler v1_1 " : S-Function  LoadFcn=xlBlockLoadCallback(gcbh);  FunctionName=sysgen  Parameters=ptable_  EnableBusSupport=off  mask(Xilinx DDS Compiler v1_1 Block){dds_clock_rate=100.0, sfdr=36.0, frequency_resolution=0.4, mode_sgadvanced=, mode=Sine, neg_sin_sgadvanced=, neg_sin=off, neg_cos_sgadvanced=, neg_cos=off, channels_sgadvanced=, channels=1, output_frequency_type_sgadvanced=, output_frequency_type=Fixed, output_frequency_array=[1.0], phase_offset_type_sgadvanced=, phase_offset_type=None, phase_offset_array=[0.0], explicit_period_sgadvanced=, explicit_period=on, period=1, noise_shaping_sgadvanced=, noise_shaping=None, channel_port_sgadvanced=, channel_port=off, RFD_sgadvanced=, RFD=off, RDY_sgadvanced=, RDY=off, rst_sgadvanced=, rst=off, en_sgadvanced=, en=on, dbl_ovrd_sgadvanced=, dbl_ovrd=off, mem_type_sgadvanced=, mem_type=Distributed Memory, dsp48_use_sgadvanced=, dsp48_use=Minimal, latency_configuration_sgadvanced=, latency_configuration=Auto, latency=1, accum_latency_sgadvanced=, accum_latency=One Cycle, xl_use_area_sgadvanced=, xl_use_area=off, xl_area=[0,0,0,0,0,0,0], version=1, acc_latency=2, has_advanced_control=0, sggui_pos=-1,-1,-1,-1, block_type=dds_compilerv11, block_version=, sg_icon_stat=60,60,-1,-1,white,blue,0,07734,right,,[ ],[ ], sg_mask_display=|, sg_list_contents=, sg_blockgui_xml=}
      mask sg_mask_display=|
      | fprintf('','COMMENT: begin icon graphics');
      | patch([0 60 60 0 0 ],[0 0 60 60 0 ],[0.77 0.82 0.91 ]);
      | plot([0 60 60 0 0 ],[0 0 60 60 0 ]);
      | patch([12.2 23.76 31.76 39.76 47.76 31.76 20.2 12.2 ],[38.88 38.88 46.88 38.88 46.88 46.88 46.88 38.88 ],[1 1 1 ]);
      | patch([20.2 31.76 23.76 12.2 20.2 ],[30.88 30.88 38.88 38.88 30.88 ],[0.931 0.946 0.973 ]);
      | patch([12.2 23.76 31.76 20.2 12.2 ],[22.88 22.88 30.88 30.88 22.88 ],[1 1 1 ]);
      | patch([20.2 47.76 39.76 31.76 23.76 12.2 20.2 ],[14.88 14.88 22.88 14.88 22.88 22.88 14.88 ],[0.931 0.946 0.973 ]);
      | fprintf('','COMMENT: end icon graphics');
      | fprintf('','COMMENT: begin icon text');
      | fprintf('','COMMENT: end icon text');
      mask prompts: dds_clock_rate "DDS clock rate (MHz)"; sfdr "Spurious free dynamic range (dB)"; frequency_resolution "Frequency resolution (Hz)"; mode_sgadvanced ""; mode "Function"; neg_sin_sgadvanced ""; neg_sin "Negative sine"; neg_cos_sgadvanced ""; neg_cos "Negative cosine"; channels_sgadvanced ""; output_frequency_type_sgadvanced ""; output_frequency_type "Type"; output_frequency_array "Output frequency array (MHz)"; phase_offset_type_sgadvanced ""; phase_offset_type "Type"; phase_offset_array "Phase offset angle array (x 2pi Radians)"; explicit_period_sgadvanced ""; explicit_period "Sample period source"; period "Explicit period"; noise_shaping_sgadvanced ""; noise_shaping "Noise Shaping"; channel_port_sgadvanced ""; channel_port "Provide channel port"; RFD_sgadvanced ""; RFD "Provide rfd port"; RDY_sgadvanced ""; RDY "Provide rdy port"; rst_sgadvanced ""; rst "Provide synchronous reset port"; en_sgadvanced ""; en "Provide enable port"; dbl_ovrd_sgadvanced ""; dbl_ovrd "Override with doubles"; mem_type_sgadvanced ""; mem_type "Memory type"; dsp48_use_sgadvanced ""; dsp48_use "DSP48 Use"; latency_configuration_sgadvanced ""; latency_configuration "Latency configuration"; accum_latency_sgadvanced ""; accum_latency "Accumulator latency"; xl_use_area_sgadvanced ""; xl_use_area "Define FPGA area for resource estimation"; xl_area "FPGA area [slices, FFs, BRAMs, LUTs, IOBs, emb. mults, TBUFs]"; version ""; acc_latency ""; has_advanced_control ""; sggui_pos ""; block_type ""; block_version ""; sg_icon_stat ""; sg_mask_display ""; sg_list_contents ""; sg_blockgui_xml ""
      mask help: Xilinx DDS Compiler v1_1
      mask init:
      | try
      |   tmp_gcb = gcb;
      |   tmp_gcbh = gcbh;
      |   if (strcmp('SysGenIndex',get_param(bdroot(tmp_gcbh),'tag')) && ~isempty(regexp(bdroot(tmp_gcb), '^xbs', 'once')))
      |     return;
      |   end;
      |   xlMungeMaskParams;
      |   block_config = 'sysgen_blockset:Removed_config';
      | 
      |   block_type='dds_compilerv11';
      | nport = get_param(gcbh, 'ports');
      | nin = nport(1);
      | nout = nport(2);
      | 
      |   serialized_declarations = '{''RDY''=>''Int'',''RFD''=>''Int'',''accum_latency''=>''Int'',''channel_port''=>''Int'',''channels''=>''Int'',''dds_clock_rate''=>''Double'',''dsp48_use''=>''Int'',''en''=>''Int'',''explicit_period''=>''Int'',''frequency_resolution''=>''Double'',''latency''=>''Int'',''latency_configuration''=>''Int'',''mem_type''=>''Int'',''mode''=>''Int'',''neg_cos''=>''Int'',''neg_sin''=>''Int'',''noise_shaping''=>''Int'',''output_frequency_array''=>''DoubleVector'',''output_frequency_type''=>''Int'',''period''=>''Double'',''phase_offset_array''=>''DoubleVector'',''phase_offset_type''=>''Int'',''rst''=>''Int'',''sfdr''=>''Double'',''version''=>''Int'',''block_type''=>''String'',''nin''=>''Double'',''nout''=>''Double''}';
      |   ptable_ = xlblockprep(get_param(tmp_gcb, 'MaskWSVariables'));
      |   try
      |     xlBlockMoveCallback(tmp_gcbh);
      |   catch 
      |      clear global xl_updateicon_recursion_guard;
      |   end;
      | catch
      |   global dbgsysgen;
      |   if(~isempty(dbgsysgen) && dbgsysgen)
      |     e = regexprep(lasterr, '\n', '\nError: ');
      |     disp(['Error: While running MaskInit code on block ' tmp_gcb ': ' e]);
      |     error(e);
      |   end
      | end
      settings: CopyFcn=xlBlockMoveCallback(gcbh);  DeleteFcn=xlDestroyGui(gcbh);  ModelCloseFcn=xlDestroyGui(gcbh);  PreSaveFcn=xlBlockPreSaveCallback(gcbh);  PostSaveFcn=xlBlockPostSaveCallback(gcbh);  DestroyFcn=xlDestroyGui(gcbh);  OpenFcn=xlOpenGui(gcbh, 'ddscompiler10_gui.xml', @xlremovedenablement, -1)  CloseFcn=xlDestroyGui(gcbh);  MoveFcn=xlBlockMoveCallback(gcbh);
      mask Help: eval('');xlDoc('-book','sysgen','-topic','DDS_Compiler_v1_1');
      mask StyleString: edit,edit,edit,edit,popup(Sine|Cosine|Sine and Cosine),edit,checkbox,edit,checkbox,edit,popup(1|2|3|4|5|6|7|8|9|10|11|12|13|14|15|16),edit,popup(Fixed|Programmable),edit,edit,popup(Fixed|Programmable|None),edit,edit,popup(on|off),edit,edit,popup(None|Phase dithering|Taylor series corrected|Auto),edit,checkbox,edit,checkbox,edit,checkbox,edit,checkbox,edit,checkbox,edit,checkbox,edit,popup(Distributed Memory|Block RAM),edit,popup(Minimal|Maximal),edit,popup(Auto|Configurable),edit,edit,popup(Zero Cycle|One Cycle),edit,checkbox,edit,edit,edit,edit,edit,edit,edit,edit,edit,edit,edit
      mask Display:
      | fprintf('','COMMENT: begin icon graphics');
      | patch([0 60 60 0 0 ],[0 0 60 60 0 ],[0.77 0.82 0.91 ]);
      | plot([0 60 60 0 0 ],[0 0 60 60 0 ]);
      | patch([12.2 23.76 31.76 39.76 47.76 31.76 20.2 12.2 ],[38.88 38.88 46.88 38.88 46.88 46.88 46.88 38.88 ],[1 1 1 ]);
      | patch([20.2 31.76 23.76 12.2 20.2 ],[30.88 30.88 38.88 38.88 30.88 ],[0.931 0.946 0.973 ]);
      | patch([12.2 23.76 31.76 20.2 12.2 ],[22.88 22.88 30.88 30.88 22.88 ],[1 1 1 ]);
      | patch([20.2 47.76 39.76 31.76 23.76 12.2 20.2 ],[14.88 14.88 22.88 14.88 22.88 22.88 14.88 ],[0.931 0.946 0.973 ]);
      | fprintf('','COMMENT: end icon graphics');
      | fprintf('','COMMENT: begin icon text');
      | fprintf('','COMMENT: end icon text');
  "DDS Compiler v2_0 " : S-Function  LoadFcn=xlBlockLoadCallback(gcbh);  FunctionName=sysgen  Parameters=ptable_  EnableBusSupport=off  mask(Xilinx DDS Compiler v2_0 Block){dds_clock_rate=100.0, sfdr=36.0, frequency_resolution=0.4, mode_sgadvanced=, mode=Sine, neg_sin_sgadvanced=, neg_sin=off, neg_cos_sgadvanced=, neg_cos=off, channels_sgadvanced=, channels=1, output_frequency_type_sgadvanced=, output_frequency_type=Fixed, output_frequency_array=[1.0], phase_offset_type_sgadvanced=, phase_offset_type=None, phase_offset_array=[0.0], explicit_period_sgadvanced=, explicit_period=on, period=1, noise_shaping_sgadvanced=, noise_shaping=None, channel_port_sgadvanced=, channel_port=off, RFD_sgadvanced=, RFD=off, RDY_sgadvanced=, RDY=off, rst_sgadvanced=, rst=off, en_sgadvanced=, en=on, dbl_ovrd_sgadvanced=, dbl_ovrd=off, mem_type_sgadvanced=, mem_type=Block RAM, dsp48_use_sgadvanced=, dsp48_use=Minimal, latency_configuration_sgadvanced=, latency_configuration=Auto, latency=1, accum_latency_sgadvanced=, accum_latency=One Cycle, xl_use_area_sgadvanced=, xl_use_area=off, xl_area=[0,0,0,0,0,0,0], version=1, acc_latency=2, has_advanced_control=0, sggui_pos=-1,-1,-1,-1, block_type=dds_compilerv20, block_version=, sg_icon_stat=60,60,-1,-1,white,blue,0,07734,right,,[ ],[ ], sg_mask_display=|, sg_list_contents=, sg_blockgui_xml=}
      mask sg_mask_display=|
      | fprintf('','COMMENT: begin icon graphics');
      | patch([0 60 60 0 0 ],[0 0 60 60 0 ],[0.77 0.82 0.91 ]);
      | plot([0 60 60 0 0 ],[0 0 60 60 0 ]);
      | patch([12.2 23.76 31.76 39.76 47.76 31.76 20.2 12.2 ],[38.88 38.88 46.88 38.88 46.88 46.88 46.88 38.88 ],[1 1 1 ]);
      | patch([20.2 31.76 23.76 12.2 20.2 ],[30.88 30.88 38.88 38.88 30.88 ],[0.931 0.946 0.973 ]);
      | patch([12.2 23.76 31.76 20.2 12.2 ],[22.88 22.88 30.88 30.88 22.88 ],[1 1 1 ]);
      | patch([20.2 47.76 39.76 31.76 23.76 12.2 20.2 ],[14.88 14.88 22.88 14.88 22.88 22.88 14.88 ],[0.931 0.946 0.973 ]);
      | fprintf('','COMMENT: end icon graphics');
      | fprintf('','COMMENT: begin icon text');
      | fprintf('','COMMENT: end icon text');
      mask prompts: dds_clock_rate "DDS clock rate (MHz)"; sfdr "Spurious free dynamic range (dB)"; frequency_resolution "Frequency resolution (Hz)"; mode_sgadvanced ""; mode "Function"; neg_sin_sgadvanced ""; neg_sin "Negative sine"; neg_cos_sgadvanced ""; neg_cos "Negative cosine"; channels_sgadvanced ""; output_frequency_type_sgadvanced ""; output_frequency_type "Type"; output_frequency_array "Output frequency array (MHz)"; phase_offset_type_sgadvanced ""; phase_offset_type "Type"; phase_offset_array "Phase offset angle array (x 2pi Radians)"; explicit_period_sgadvanced ""; explicit_period "Sample period source"; period "Explicit period"; noise_shaping_sgadvanced ""; noise_shaping "Noise Shaping"; channel_port_sgadvanced ""; channel_port "Provide channel port"; RFD_sgadvanced ""; RFD "Provide rfd port"; RDY_sgadvanced ""; RDY "Provide rdy port"; rst_sgadvanced ""; rst "Provide synchronous reset port"; en_sgadvanced ""; en "Provide enable port"; dbl_ovrd_sgadvanced ""; dbl_ovrd "Override with doubles"; mem_type_sgadvanced ""; mem_type "Memory type"; dsp48_use_sgadvanced ""; dsp48_use "DSP48 Use"; latency_configuration_sgadvanced ""; latency_configuration "Latency configuration"; accum_latency_sgadvanced ""; accum_latency "Accumulator latency"; xl_use_area_sgadvanced ""; xl_use_area "Define FPGA area for resource estimation"; xl_area "FPGA area [slices, FFs, BRAMs, LUTs, IOBs, emb. mults, TBUFs]"; version ""; acc_latency ""; has_advanced_control ""; sggui_pos ""; block_type ""; block_version ""; sg_icon_stat ""; sg_mask_display ""; sg_list_contents ""; sg_blockgui_xml ""
      mask help: Xilinx DDS Compiler v2_0
      mask init:
      | try
      |   tmp_gcb = gcb;
      |   tmp_gcbh = gcbh;
      |   if (strcmp('SysGenIndex',get_param(bdroot(tmp_gcbh),'tag')) && ~isempty(regexp(bdroot(tmp_gcb), '^xbs', 'once')))
      |     return;
      |   end;
      |   xlMungeMaskParams;
      |   block_config = 'sysgen_blockset:Removed_config';
      | 
      |   block_type='dds_compilerv20';
      | nport = get_param(gcbh, 'ports');
      | nin = nport(1);
      | nout = nport(2);
      | 
      |   serialized_declarations = '{''RDY''=>''Int'',''RFD''=>''Int'',''accum_latency''=>''Int'',''channel_port''=>''Int'',''channels''=>''Int'',''dds_clock_rate''=>''Double'',''dsp48_use''=>''Int'',''en''=>''Int'',''explicit_period''=>''Int'',''frequency_resolution''=>''Double'',''latency''=>''Int'',''latency_configuration''=>''Int'',''mem_type''=>''Int'',''mode''=>''Int'',''neg_cos''=>''Int'',''neg_sin''=>''Int'',''noise_shaping''=>''Int'',''output_frequency_array''=>''DoubleVector'',''output_frequency_type''=>''Int'',''period''=>''Double'',''phase_offset_array''=>''DoubleVector'',''phase_offset_type''=>''Int'',''rst''=>''Int'',''sfdr''=>''Double'',''version''=>''Int'',''block_type''=>''String'',''nin''=>''Double'',''nout''=>''Double''}';
      |   ptable_ = xlblockprep(get_param(tmp_gcb, 'MaskWSVariables'));
      |   try
      |     xlBlockMoveCallback(tmp_gcbh);
      |   catch 
      |      clear global xl_updateicon_recursion_guard;
      |   end;
      | catch
      |   global dbgsysgen;
      |   if(~isempty(dbgsysgen) && dbgsysgen)
      |     e = regexprep(lasterr, '\n', '\nError: ');
      |     disp(['Error: While running MaskInit code on block ' tmp_gcb ': ' e]);
      |     error(e);
      |   end
      | end
      settings: CopyFcn=xlBlockMoveCallback(gcbh);  DeleteFcn=xlDestroyGui(gcbh);  ModelCloseFcn=xlDestroyGui(gcbh);  PreSaveFcn=xlBlockPreSaveCallback(gcbh);  PostSaveFcn=xlBlockPostSaveCallback(gcbh);  DestroyFcn=xlDestroyGui(gcbh);  OpenFcn=xlOpenGui(gcbh, 'ddscompiler20_gui.xml', @xlremovedenablement, -1)  CloseFcn=xlDestroyGui(gcbh);  MoveFcn=xlBlockMoveCallback(gcbh);
      mask Help: eval('');xlDoc('-book','sysgen','-topic','DDS_Compiler_v2_0');
      mask StyleString: edit,edit,edit,edit,popup(Sine|Cosine|Sine and Cosine),edit,checkbox,edit,checkbox,edit,popup(1|2|3|4|5|6|7|8|9|10|11|12|13|14|15|16),edit,popup(Fixed|Programmable),edit,edit,popup(Fixed|Programmable|None),edit,edit,popup(on|off),edit,edit,popup(None|Phase dithering|Taylor series corrected|Auto),edit,checkbox,edit,checkbox,edit,checkbox,edit,checkbox,edit,checkbox,edit,checkbox,edit,popup(Distributed Memory|Block RAM),edit,popup(Minimal|Maximal),edit,popup(Auto|Configurable),edit,edit,popup(Zero Cycle|One Cycle),edit,checkbox,edit,edit,edit,edit,edit,edit,edit,edit,edit,edit,edit
      mask Display:
      | fprintf('','COMMENT: begin icon graphics');
      | patch([0 60 60 0 0 ],[0 0 60 60 0 ],[0.77 0.82 0.91 ]);
      | plot([0 60 60 0 0 ],[0 0 60 60 0 ]);
      | patch([12.2 23.76 31.76 39.76 47.76 31.76 20.2 12.2 ],[38.88 38.88 46.88 38.88 46.88 46.88 46.88 38.88 ],[1 1 1 ]);
      | patch([20.2 31.76 23.76 12.2 20.2 ],[30.88 30.88 38.88 38.88 30.88 ],[0.931 0.946 0.973 ]);
      | patch([12.2 23.76 31.76 20.2 12.2 ],[22.88 22.88 30.88 30.88 22.88 ],[1 1 1 ]);
      | patch([20.2 47.76 39.76 31.76 23.76 12.2 20.2 ],[14.88 14.88 22.88 14.88 22.88 22.88 14.88 ],[0.931 0.946 0.973 ]);
      | fprintf('','COMMENT: end icon graphics');
      | fprintf('','COMMENT: begin icon text');
      | fprintf('','COMMENT: end icon text');
  "DDS v4_0 " : S-Function  LoadFcn=xlBlockLoadCallback(gcbh);  FunctionName=sysgen  Parameters=ptable_  EnableBusSupport=off  mask(Xilinx Direct Digital Synthesizer v4_0 Block){mode_sgadvanced=, mode=Sine, neg_sin_sgadvanced=, neg_sin=off, neg_cos_sgadvanced=, neg_cos=off, n_bits=32, phase_increment_type_sgadvanced=, phase_increment_type=Constant, phase_increment=1/10, phase_offset_type_sgadvanced=, phase_offset_type=None, phase_offset=1/4, rst_sgadvanced=, rst=off, en_sgadvanced=, en=on, lut_addr_bits=10, acc_latency_sgadvanced=, acc_latency=One Cycle, acc_n_bits=32, phase_dithering_sgadvanced=, phase_dithering=off, dbl_ovrd_sgadvanced=, dbl_ovrd=off, explicit_period_sgadvanced=, explicit_period=off, period=1, mem_type_sgadvanced=, mem_type=Distributed Memory, pipeline_sgadvanced=, pipeline=off, use_rpm_sgadvanced=, use_rpm=off, xl_use_area_sgadvanced=, xl_use_area=off, xl_area=[0,0,0,0,0,0,0], has_advanced_control=0, sggui_pos=-1,-1,-1,-1, block_type=ddsv4, block_version=, sg_icon_stat=55,60,-1,-1,white,blue,0,07734,right,,[ ],[ ], sg_mask_display=|, sg_list_contents=, sg_blockgui_xml=}
      mask sg_mask_display=|
      | fprintf('','COMMENT: begin icon graphics');
      | patch([0 55 55 0 0 ],[0 0 60 60 0 ],[0.77 0.82 0.91 ]);
      | plot([0 55 55 0 0 ],[0 0 60 60 0 ]);
      | patch([11.425 21.54 28.54 35.54 42.54 28.54 18.425 11.425 ],[37.77 37.77 44.77 37.77 44.77 44.77 44.77 37.77 ],[1 1 1 ]);
      | patch([18.425 28.54 21.54 11.425 18.425 ],[30.77 30.77 37.77 37.77 30.77 ],[0.931 0.946 0.973 ]);
      | patch([11.425 21.54 28.54 18.425 11.425 ],[23.77 23.77 30.77 30.77 23.77 ],[1 1 1 ]);
      | patch([18.425 42.54 35.54 28.54 21.54 11.425 18.425 ],[16.77 16.77 23.77 16.77 23.77 23.77 16.77 ],[0.931 0.946 0.973 ]);
      | fprintf('','COMMENT: end icon graphics');
      | fprintf('','COMMENT: begin icon text');
      | fprintf('','COMMENT: end icon text');
      mask prompts: mode_sgadvanced ""; mode "Function"; neg_sin_sgadvanced ""; neg_sin "Negative sine"; neg_cos_sgadvanced ""; neg_cos "Negative cosine"; n_bits "Output width"; phase_increment_type_sgadvanced ""; phase_increment_type "Type"; phase_increment "Normalized phase increment  (cycles per sample)"; phase_offset_type_sgadvanced ""; phase_offset_type "Type"; phase_offset "Normalized phase offset  (cycles per sample)"; rst_sgadvanced ""; rst "Provide synchronous reset port"; en_sgadvanced ""; en "Provide enable port"; lut_addr_bits "Lookup table input width"; acc_latency_sgadvanced ""; acc_latency "Accumulator latency"; acc_n_bits "Accumulator width"; phase_dithering_sgadvanced ""; phase_dithering "Use phase dithering"; dbl_ovrd_sgadvanced ""; dbl_ovrd "Override with doubles"; explicit_period_sgadvanced ""; explicit_period "Specify explicit sample period"; period ""; mem_type_sgadvanced ""; mem_type "Memory type"; pipeline_sgadvanced ""; pipeline "Pipeline for maximum performance"; use_rpm_sgadvanced ""; use_rpm "Use core placement information"; xl_use_area_sgadvanced ""; xl_use_area "Define FPGA area for resource estimation"; xl_area "FPGA area [slices, FFs, BRAMs, LUTs, IOBs, emb. mults, TBUFs]"; has_advanced_control ""; sggui_pos ""; block_type ""; block_version ""; sg_icon_stat ""; sg_mask_display ""; sg_list_contents ""; sg_blockgui_xml ""
      mask help: Xilinx Direct Digital Synthesizer v4_0
      mask init:
      | try
      |   tmp_gcb = gcb;
      |   tmp_gcbh = gcbh;
      |   if (strcmp('SysGenIndex',get_param(bdroot(tmp_gcbh),'tag')) && ~isempty(regexp(bdroot(tmp_gcb), '^xbs', 'once')))
      |     return;
      |   end;
      |   xlMungeMaskParams;
      |   block_config = 'sysgen_blockset:Removed_config';
      | 
      |   block_type='ddsv4';
      | nport = get_param(gcbh, 'ports');
      | nin = nport(1);
      | nout = nport(2);
      | 
      |   serialized_declarations = '{''acc_latency''=>''Int'',''acc_n_bits''=>''Int'',''accwidth''=>''Int'',''bin_pt''=>''Int'',''lut_addr_bits''=>''Int'',''memtype''=>''Int'',''mode''=>''Int'',''n_bits''=>''Int'',''neg_cos''=>''Int'',''neg_sin''=>''Int'',''pd''=>''Int'',''period''=>''Double'',''phase_angle_width''=>''Int'',''phase_inc''=>''Double'',''phase_increment_type''=>''Int'',''phase_offset''=>''Double'',''phase_offset_type''=>''Int'',''pipelined''=>''Int'',''pitype''=>''Int'',''potype''=>''Int'',''use_rpm''=>''Int'',''block_type''=>''String'',''nin''=>''Double'',''nout''=>''Double''}';
      |   xlddsv4_init();
      |   ptable_ = xlblockprep(get_param(tmp_gcb, 'MaskWSVariables'));
      |   try
      |     xlBlockMoveCallback(tmp_gcbh);
      |   catch 
      |      clear global xl_updateicon_recursion_guard;
      |   end;
      | catch
      |   global dbgsysgen;
      |   if(~isempty(dbgsysgen) && dbgsysgen)
      |     e = regexprep(lasterr, '\n', '\nError: ');
      |     disp(['Error: While running MaskInit code on block ' tmp_gcb ': ' e]);
      |     error(e);
      |   end
      | end
      settings: CopyFcn=xlBlockMoveCallback(gcbh);  DeleteFcn=xlDestroyGui(gcbh);  ModelCloseFcn=xlDestroyGui(gcbh);  PreSaveFcn=xlBlockPreSaveCallback(gcbh);  PostSaveFcn=xlBlockPostSaveCallback(gcbh);  DestroyFcn=xlDestroyGui(gcbh);  OpenFcn=xlOpenGui(gcbh, 'ddsv4_gui.xml', @xlremovedenablement, -1)  CloseFcn=xlDestroyGui(gcbh);  MoveFcn=xlBlockMoveCallback(gcbh);
      mask Help: eval('');xlDoc('-book','sysgen','-topic','DDS_v4_0');
      mask StyleString: edit,popup(Sine|Cosine|Sine and Cosine),edit,checkbox,edit,checkbox,edit,edit,popup(Constant|Register),edit,edit,popup(Constant|Register|None),edit,edit,checkbox,edit,checkbox,edit,edit,popup(Zero Cycle|One Cycle),edit,edit,checkbox,edit,checkbox,edit,checkbox,edit,edit,popup(Distributed Memory|Block RAM),edit,checkbox,edit,checkbox,edit,checkbox,edit,edit,edit,edit,edit,edit,edit,edit,edit
      mask Display:
      | fprintf('','COMMENT: begin icon graphics');
      | patch([0 55 55 0 0 ],[0 0 60 60 0 ],[0.77 0.82 0.91 ]);
      | plot([0 55 55 0 0 ],[0 0 60 60 0 ]);
      | patch([11.425 21.54 28.54 35.54 42.54 28.54 18.425 11.425 ],[37.77 37.77 44.77 37.77 44.77 44.77 44.77 37.77 ],[1 1 1 ]);
      | patch([18.425 28.54 21.54 11.425 18.425 ],[30.77 30.77 37.77 37.77 30.77 ],[0.931 0.946 0.973 ]);
      | patch([11.425 21.54 28.54 18.425 11.425 ],[23.77 23.77 30.77 30.77 23.77 ],[1 1 1 ]);
      | patch([18.425 42.54 35.54 28.54 21.54 11.425 18.425 ],[16.77 16.77 23.77 16.77 23.77 23.77 16.77 ],[0.931 0.946 0.973 ]);
      | fprintf('','COMMENT: end icon graphics');
      | fprintf('','COMMENT: begin icon text');
      | fprintf('','COMMENT: end icon text');
